simulink model "electrotac_feedback_emg_2016a"  (R2016a)
settings: Solver=FixedStepDiscrete  StartTime=0.0  StopTime=inf  FixedStep=0.02  RelTol=1e-3
undefined symbols (not defined in the file): DiscIntNeverNeededParam
libraries: PowermateLibrary x1, LIB_RehaMove3 x1, STIMYOLibrary x1
(part 2 of 3)

== stateflow chart electrotac_feedback_emg_2016a/stim_chart ==
  state preview
    state force_feedback1
      entry:
      reset_integrator = 0;
      during:
      stim_off_pw= [1 1 1 1];
      force_feedback_input = emg_value/12;
      state stim_n
        state stim_on
          during:
          pulsewidth = func.commonElectrode_4ch_stim(th_max,th_min,def_current,-def_current/4,0,'n','pw');
          current = func.commonElectrode_4ch_stim(th_max,th_min,def_current,-def_current/4,0,'n','cr');
          stim_status = func.commonElectrode_4ch_stim(th_max,th_min,def_current,-def_current/4,0,'n','lg');
          %ch3
        state stim_off [commented out]
          during:
          pulsewidth = func.commonElectrode_4ch_stim([0 0 0 0],th_min,def_current,-def_current/4,0,'e','pw');
          current = func.commonElectrode_4ch_stim([0 0 0 0],th_min,def_current,-def_current/4,0,'e','cr');
          %ch3
        (default) -> preview.force_feedback1.stim_n.stim_on
        preview.force_feedback1.stim_n.stim_on -> preview.force_feedback1.stim_n.stim_off [commented out] : after(input_freq,sec)
        preview.force_feedback1.stim_n.stim_off -> preview.force_feedback1.stim_n.stim_on [commented out] : after(input_freq,sec)
      state pos_nw6
        state stim_on
          during:
          pulsewidth = func.commonElectrode_4ch_stim(th_max,th_min,def_current,-def_current/4,0,'nw','pw');
          current = func.commonElectrode_4ch_stim(th_max,th_min,def_current,-def_current/4,0,'nw','cr');
          stim_status = func.commonElectrode_4ch_stim(th_max,th_min,def_current,-def_current/4,0,'nw','lg');
          %ch3
        state stim_off
          during:
          pulsewidth = func.commonElectrode_4ch_stim(stim_off_pw,th_min,def_current,-def_current/4,0,'nw','pw');
          current = func.commonElectrode_4ch_stim(stim_off_pw,th_min,def_current,-def_current/4,0,'nw','cr');
          stim_status = func.commonElectrode_4ch_stim(stim_off_pw,th_min,def_current,-def_current/4,0,'nw','lg');
          %ch3
        (default) -> preview.force_feedback1.pos_nw6.stim_on
        preview.force_feedback1.pos_nw6.stim_on -> preview.force_feedback1.pos_nw6.stim_off : after(0.2,sec)
        preview.force_feedback1.pos_nw6.stim_off -> preview.force_feedback1.pos_nw6.stim_on : after(0.2,sec)
      state pos_nw9
        state stim_on
          during:
          pulsewidth = func.commonElectrode_4ch_stim(th_max,th_min,def_current,-def_current/4,0,'ne','pw');
          current = func.commonElectrode_4ch_stim(th_max,th_min,def_current,-def_current/4,0,'ne','cr');
          stim_status = func.commonElectrode_4ch_stim(th_max,th_min,def_current,-def_current/4,0,'ne','lg');
          %ch3
        state stim_off
          during:
          pulsewidth = func.commonElectrode_4ch_stim(stim_off_pw,th_min,def_current,-def_current/4,0,'ne','pw');
          current = func.commonElectrode_4ch_stim(stim_off_pw,th_min,def_current,-def_current/4,0,'ne','cr');
          stim_status = func.commonElectrode_4ch_stim(stim_off_pw,th_min,def_current,-def_current/4,0,'ne','lg');
          %ch3
        (default) -> preview.force_feedback1.pos_nw9.stim_on
        preview.force_feedback1.pos_nw9.stim_on -> preview.force_feedback1.pos_nw9.stim_off : after(0.2,sec)
        preview.force_feedback1.pos_nw9.stim_off -> preview.force_feedback1.pos_nw9.stim_on : after(0.2,sec)
      state pos_nw10
        state stim_on
          during:
          pulsewidth = func.commonElectrode_4ch_stim(th_max,th_min,def_current,-def_current/4,0,'e','pw');
          current = func.commonElectrode_4ch_stim(th_max,th_min,def_current,-def_current/4,0,'e','cr');
          stim_status = func.commonElectrode_4ch_stim(th_max,th_min,def_current,-def_current/4,0,'e','lg');
          %ch3
        state stim_off [commented out]
          during:
          pulsewidth = func.commonElectrode_4ch_stim(stim_off_pw,th_min,def_current,-def_current/4,0,'e','pw');
          current = func.commonElectrode_4ch_stim(stim_off_pw,th_min,def_current,-def_current/4,0,'e','cr');
          stim_status = func.commonElectrode_4ch_stim(stim_off_pw,th_min,def_current,-def_current/4,0,'e','lg');
          %ch3
        (default) -> preview.force_feedback1.pos_nw10.stim_on
        preview.force_feedback1.pos_nw10.stim_on -> preview.force_feedback1.pos_nw10.stim_off [commented out] : after(0.2,sec)
        preview.force_feedback1.pos_nw10.stim_off -> preview.force_feedback1.pos_nw10.stim_on [commented out] : after(0.2,sec)
      state forcefeedback_3
        state stim_on
          during:
          pulsewidth = func.commonElectrode_4ch_stim(th_max,th_min,def_current,-def_current/4,0,'w','pw');
          current = func.commonElectrode_4ch_stim(th_max,th_min,def_current,-def_current/4,0,'w','cr');
          stim_status = func.commonElectrode_4ch_stim(th_max,th_min,def_current,-def_current/4,0,'w','lg');
          %ch3
        state stim_off [commented out]
          during:
          pulsewidth = func.commonElectrode_4ch_stim(stim_off_pw,th_min,def_current,-def_current/4,0,'nw','pw');
          current = func.commonElectrode_4ch_stim(stim_off_pw,th_min,def_current,-def_current/4,0,'nw','cr');
          stim_status = func.commonElectrode_4ch_stim(stim_off_pw,th_min,def_current,-def_current/4,0,'nw','lg');
          %ch3
        preview.force_feedback1.forcefeedback_3.stim_on -> preview.force_feedback1.forcefeedback_3.stim_off [commented out] : after(0.2,sec)
        preview.force_feedback1.forcefeedback_3.stim_off -> preview.force_feedback1.forcefeedback_3.stim_on [commented out] : after(0.2,sec)
      state forcefeedback_2
        state stim_on
          during:
          pulsewidth = func.commonElectrode_4ch_stim(th_max,th_min,def_current,-def_current/4,0,'w','pw');
          current = func.commonElectrode_4ch_stim(th_max,th_min,def_current,-def_current/4,0,'w','cr');
          stim_status = func.commonElectrode_4ch_stim(th_max,th_min,def_current,-def_current/4,0,'w','lg');
          %ch3
        state stim_off
          during:
          pulsewidth = func.commonElectrode_4ch_stim(stim_off_pw,th_min,def_current,-def_current/4,0,'w','pw');
          current = func.commonElectrode_4ch_stim(stim_off_pw,th_min,def_current,-def_current/4,0,'w','cr');
          stim_status = func.commonElectrode_4ch_stim(stim_off_pw,th_min,def_current,-def_current/4,0,'w','lg');
          %ch3
        (default) -> preview.force_feedback1.forcefeedback_2.stim_on
        preview.force_feedback1.forcefeedback_2.stim_on -> preview.force_feedback1.forcefeedback_2.stim_off : after(0.2,sec)
        preview.force_feedback1.forcefeedback_2.stim_off -> preview.force_feedback1.forcefeedback_2.stim_on : after(0.2,sec)
      state pos_nw11
        state stim_on
          during:
          pulsewidth = func.commonElectrode_4ch_stim(th_max,th_min,def_current,-def_current/4,0,'e','pw');
          current = func.commonElectrode_4ch_stim(th_max,th_min,def_current,-def_current/4,0,'e','cr');
          stim_status = func.commonElectrode_4ch_stim(th_max,th_min,def_current,-def_current/4,0,'e','lg');
          %ch3
        state stim_off
          during:
          pulsewidth = func.commonElectrode_4ch_stim(stim_off_pw,th_min,def_current,-def_current/4,0,'e','pw');
          current = func.commonElectrode_4ch_stim(stim_off_pw,th_min,def_current,-def_current/4,0,'e','cr');
          stim_status = func.commonElectrode_4ch_stim(stim_off_pw,th_min,def_current,-def_current/4,0,'e','lg');
          %ch3
        (default) -> preview.force_feedback1.pos_nw11.stim_on
        preview.force_feedback1.pos_nw11.stim_on -> preview.force_feedback1.pos_nw11.stim_off : after(0.2,sec)
        preview.force_feedback1.pos_nw11.stim_off -> preview.force_feedback1.pos_nw11.stim_on : after(0.2,sec)
      state stim_w
        state stim_on
          during:
          pulsewidth = func.commonElectrode_4ch_stim(th_max,th_min,def_current,-def_current/4,0,'sw','pw');
          current = func.commonElectrode_4ch_stim(th_max,th_min,def_current,-def_current/4,0,'sw','cr');
          stim_status = func.commonElectrode_4ch_stim(th_max,th_min,def_current,-def_current/4,0,'sw','lg');
          %ch3
        state stim_off
          during:
          pulsewidth = func.commonElectrode_4ch_stim(stim_off_pw,th_min,def_current,-def_current/4,0,'sw','pw');
          current = func.commonElectrode_4ch_stim(stim_off_pw,th_min,def_current,-def_current/4,0,'sw','cr');
          stim_status = func.commonElectrode_4ch_stim(stim_off_pw,th_min,def_current,-def_current/4,0,'sw','lg');
          %ch3
        (default) -> preview.force_feedback1.stim_w.stim_on
        preview.force_feedback1.stim_w.stim_on -> preview.force_feedback1.stim_w.stim_off : after(0.2,sec)
        preview.force_feedback1.stim_w.stim_off -> preview.force_feedback1.stim_w.stim_on : after(0.2,sec)
      state stim_e
        state stim_on
          during:
          pulsewidth = func.commonElectrode_4ch_stim(th_max,th_min,def_current,-def_current/4,0,'se','pw');
          current = func.commonElectrode_4ch_stim(th_max,th_min,def_current,-def_current/4,0,'se','cr');
          stim_status = func.commonElectrode_4ch_stim(th_max,th_min,def_current,-def_current/4,0,'se','lg');
          %ch3
        state stim_off
          during:
          pulsewidth = func.commonElectrode_4ch_stim(stim_off_pw,th_min,def_current,-def_current/4,0,'se','pw');
          current = func.commonElectrode_4ch_stim(stim_off_pw,th_min,def_current,-def_current/4,0,'se','cr');
          stim_status = func.commonElectrode_4ch_stim(stim_off_pw,th_min,def_current,-def_current/4,0,'se','lg');
          %ch3
        (default) -> preview.force_feedback1.stim_e.stim_on
        preview.force_feedback1.stim_e.stim_on -> preview.force_feedback1.stim_e.stim_off : after(0.2,sec)
        preview.force_feedback1.stim_e.stim_off -> preview.force_feedback1.stim_e.stim_on : after(0.2,sec)
      preview.force_feedback1.stim_n -> preview.force_feedback1.pos_nw9 : [c == 24]
      preview.force_feedback1.pos_nw6 -> preview.force_feedback1.stim_n : [c == 23]
      preview.force_feedback1.forcefeedback_3 -> preview.force_feedback1.pos_nw6 : [c == 22]
      preview.force_feedback1.pos_nw9 -> preview.force_feedback1.pos_nw10 : [c == 25]
      preview.force_feedback1.forcefeedback_2 -> preview.force_feedback1.forcefeedback_3 : [c == 21]
      preview.force_feedback1.pos_nw10 -> preview.force_feedback1.pos_nw11 : [c == 26]
      preview.force_feedback1.stim_w -> preview.force_feedback1.forcefeedback_2 : [c == 20]
      preview.force_feedback1.pos_nw11 -> preview.force_feedback1.stim_e : [c == 27]
      (default) -> preview.force_feedback1.stim_w
    state hand_openclosed1
      entry: reset_integrator = 0;
      during: stim_off_pw= [1 1 1 1]
      state neutral
        state pos_west2
          during:
          pulsewidth = func.commonElectrode_4ch_stim(stim_off_pw,th_min,def_current,-def_current/4,0,'ns','pw');
          current = func.commonElectrode_4ch_stim(stim_off_pw,th_min,def_current,-def_current/4,0,'ns','cr');
          stim_status = func.commonElectrode_4ch_stim(stim_off_pw,th_min,def_current,-def_current/4,0,'ns','lg');
          %ch3
      state level1
        state pos_west1
          during:
          pulsewidth = func.commonElectrode_4ch_stim(th_max,th_min,def_current,-def_current/4,0,'ns','pw');
          current = func.commonElectrode_4ch_stim(th_max,th_min,def_current,-def_current/4,0,'ns','cr');
          stim_status = func.commonElectrode_4ch_stim(th_max,th_min,def_current,-def_current/4,0,'ns','lg');
          %ch3
        state pos_west2
          during:
          pulsewidth = func.commonElectrode_4ch_stim(stim_off_pw,th_min,def_current,-def_current/4,0,'ns','pw');
          current = func.commonElectrode_4ch_stim(stim_off_pw,th_min,def_current,-def_current/4,0,'ns','cr');
          stim_status = func.commonElectrode_4ch_stim(stim_off_pw,th_min,def_current,-def_current/4,0,'ns','lg');
          %ch3
        (default) -> preview.hand_openclosed1.level1.pos_west1
        preview.hand_openclosed1.level1.pos_west1 -> preview.hand_openclosed1.level1.pos_west2 : after(0.5,sec)
        preview.hand_openclosed1.level1.pos_west2 -> preview.hand_openclosed1.level1.pos_west1 : after(0.5,sec)
      state level2
        state pos_west1
          during:
          pulsewidth = func.commonElectrode_4ch_stim(th_max,th_min,def_current,-def_current/4,0,'ns','pw');
          current = func.commonElectrode_4ch_stim(th_max,th_min,def_current,-def_current/4,0,'ns','cr');
          stim_status = func.commonElectrode_4ch_stim(th_max,th_min,def_current,-def_current/4,0,'ns','lg');
          %ch3
        state pos_west2
          during:
          pulsewidth = func.commonElectrode_4ch_stim(stim_off_pw,th_min,def_current,-def_current/4,0,'ns','pw');
          current = func.commonElectrode_4ch_stim(stim_off_pw,th_min,def_current,-def_current/4,0,'ns','cr');
          stim_status = func.commonElectrode_4ch_stim(stim_off_pw,th_min,def_current,-def_current/4,0,'ns','lg');
          %ch3
        (default) -> preview.hand_openclosed1.level2.pos_west1
        preview.hand_openclosed1.level2.pos_west1 -> preview.hand_openclosed1.level2.pos_west2 : after(0.25,sec)
        preview.hand_openclosed1.level2.pos_west2 -> preview.hand_openclosed1.level2.pos_west1 : after(0.25,sec)
      state level3
        state pos_west1
          during:
          pulsewidth = func.commonElectrode_4ch_stim(th_max,th_min,def_current,-def_current/4,0,'ns','pw');
          current = func.commonElectrode_4ch_stim(th_max,th_min,def_current,-def_current/4,0,'ns','cr');
          stim_status = func.commonElectrode_4ch_stim(th_max,th_min,def_current,-def_current/4,0,'ns','lg');
          %ch3
        (default) -> preview.hand_openclosed1.level3.pos_west1
      (default) -> preview.hand_openclosed1.neutral
      preview.hand_openclosed1.neutral -> preview.hand_openclosed1.level1 [order 1] : [c == 12]
      preview.hand_openclosed1.level1 -> preview.hand_openclosed1.neutral [order 2] : [c == 17]
      preview.hand_openclosed1.level1 -> preview.hand_openclosed1.level2 [order 1] : [c == 13]
      preview.hand_openclosed1.level2 -> preview.hand_openclosed1.level1 [order 2] : [c == 16]
      preview.hand_openclosed1.level2 -> preview.hand_openclosed1.level3 [order 1] : [c == 14]
      preview.hand_openclosed1.level3 -> preview.hand_openclosed1.level2 : [c == 15]
    state handposition_map2
      entry:
      reset_integrator = 0;
      during: stim_off_pw= [1 1 1 1]
      state pos_north_e2
        during:
        pulsewidth = func.commonElectrode_4ch_stim(th_max,th_min,def_current,-def_current/4,0,'n','pw');
        current = func.commonElectrode_4ch_stim(th_max,th_min,def_current,-def_current/4,0,'n','cr');
        stim_status = func.commonElectrode_4ch_stim(th_max,th_min,def_current,-def_current/4,0,'n','lg');
        %ch1
      state pos_nw1
        state pos_west1
          during:
          pulsewidth = func.commonElectrode_4ch_stim(th_max,th_min,def_current,-def_current/4,0,'ne','pw');
          current = func.commonElectrode_4ch_stim(th_max,th_min,def_current,-def_current/4,0,'ne','cr');
          stim_status = func.commonElectrode_4ch_stim(th_max,th_min,def_current,-def_current/4,0,'ne','lg');
          %ch3
        state pos_west2
          during:
          pulsewidth = func.commonElectrode_4ch_stim(stim_off_pw,th_min,def_current,-def_current/4,0,'ne','pw');
          current = func.commonElectrode_4ch_stim(stim_off_pw,th_min,def_current,-def_current/4,0,'ne','cr');
          stim_status = func.commonElectrode_4ch_stim(stim_off_pw,th_min,def_current,-def_current/4,0,'ne','lg');
          %ch3
        (default) -> preview.handposition_map2.pos_nw1.pos_west1
        preview.handposition_map2.pos_nw1.pos_west1 -> preview.handposition_map2.pos_nw1.pos_west2 : after(0.25,sec)
        preview.handposition_map2.pos_nw1.pos_west2 -> preview.handposition_map2.pos_nw1.pos_west1 : after(0.25,sec)
      state pos_nw
        state pos_west1
          during:
          pulsewidth = func.commonElectrode_4ch_stim(th_max,th_min,def_current,-def_current/4,0,'nw','pw');
          current = func.commonElectrode_4ch_stim(th_max,th_min,def_current,-def_current/4,0,'nw','cr');
          stim_status = func.commonElectrode_4ch_stim(th_max,th_min,def_current,-def_current/4,0,'nw','lg');
          %ch3
        state pos_west2
          during:
          pulsewidth = func.commonElectrode_4ch_stim(stim_off_pw,th_min,def_current,-def_current/4,0,'nw','pw');
          current = func.commonElectrode_4ch_stim(stim_off_pw,th_min,def_current,-def_current/4,0,'nw','cr');
          stim_status = func.commonElectrode_4ch_stim(stim_off_pw,th_min,def_current,-def_current/4,0,'nw','lg');
          %ch3
        (default) -> preview.handposition_map2.pos_nw.pos_west1
        preview.handposition_map2.pos_nw.pos_west1 -> preview.handposition_map2.pos_nw.pos_west2 : after(0.25,sec)
        preview.handposition_map2.pos_nw.pos_west2 -> preview.handposition_map2.pos_nw.pos_west1 : after(0.25,sec)
      state pos_west
        during:
        pulsewidth = func.commonElectrode_4ch_stim(th_max,th_min,def_current,-def_current/4,0,'w','pw');
        current = func.commonElectrode_4ch_stim(th_max,th_min,def_current,-def_current/4,0,'w','cr');
        stim_status = func.commonElectrode_4ch_stim(th_max,th_min,def_current,-def_current/4,0,'w','lg');
        %ch3
      state pos_east
        during:
        pulsewidth = func.commonElectrode_4ch_stim(th_max,th_min,def_current,-def_current/4,0,'e','pw');
        current = func.commonElectrode_4ch_stim(th_max,th_min,def_current,-def_current/4,0,'e','cr');
        stim_status = func.commonElectrode_4ch_stim(th_max,th_min,def_current,-def_current/4,0,'e','lg');
        %ch4
      state pos_nw2
        state pos_west1
          during:
          pulsewidth = func.commonElectrode_4ch_stim(th_max,th_min,def_current,-def_current/4,0,'sw','pw');
          current = func.commonElectrode_4ch_stim(th_max,th_min,def_current,-def_current/4,0,'sw','cr');
          stim_status = func.commonElectrode_4ch_stim(th_max,th_min,def_current,-def_current/4,0,'sw','lg');
          %ch3
        state pos_west2
          during:
          pulsewidth = func.commonElectrode_4ch_stim(stim_off_pw,th_min,def_current,-def_current/4,0,'sw','pw');
          current = func.commonElectrode_4ch_stim(stim_off_pw,th_min,def_current,-def_current/4,0,'sw','cr');
          stim_status = func.commonElectrode_4ch_stim(stim_off_pw,th_min,def_current,-def_current/4,0,'sw','lg');
          %ch3
        (default) -> preview.handposition_map2.pos_nw2.pos_west1
        preview.handposition_map2.pos_nw2.pos_west1 -> preview.handposition_map2.pos_nw2.pos_west2 : after(0.25,sec)
        preview.handposition_map2.pos_nw2.pos_west2 -> preview.handposition_map2.pos_nw2.pos_west1 : after(0.25,sec)
      state pos_nw3
        state pos_west1
          during:
          pulsewidth = func.commonElectrode_4ch_stim(th_max,th_min,def_current,-def_current/4,0,'se','pw');
          current = func.commonElectrode_4ch_stim(th_max,th_min,def_current,-def_current/4,0,'se','cr');
          stim_status = func.commonElectrode_4ch_stim(th_max,th_min,def_current,-def_current/4,0,'se','lg');
          %ch3
        state pos_west2
          during:
          pulsewidth = func.commonElectrode_4ch_stim(stim_off_pw,th_min,def_current,-def_current/4,0,'e','pw');
          current = func.commonElectrode_4ch_stim(stim_off_pw,th_min,def_current,-def_current/4,0,'e','cr');
          stim_status = func.commonElectrode_4ch_stim(stim_off_pw,th_min,def_current,-def_current/4,0,'e','lg');
          %ch3
        (default) -> preview.handposition_map2.pos_nw3.pos_west1
        preview.handposition_map2.pos_nw3.pos_west1 -> preview.handposition_map2.pos_nw3.pos_west2 : after(0.25,sec)
        preview.handposition_map2.pos_nw3.pos_west2 -> preview.handposition_map2.pos_nw3.pos_west1 : after(0.25,sec)
      state pos_south_e4
        during:
        pulsewidth = func.commonElectrode_4ch_stim(th_max,th_min,def_current,-def_current/4,0,'s','pw');
        current = func.commonElectrode_4ch_stim(th_max,th_min,def_current,-def_current/4,0,'s','cr');
        stim_status = func.commonElectrode_4ch_stim(th_max,th_min,def_current,-def_current/4,0,'s','lg');
        %ch2
      (default) -> preview.handposition_map2.pos_north_e2
      preview.handposition_map2.pos_north_e2 -> preview.handposition_map2.pos_nw : [c == 3]
      preview.handposition_map2.pos_east -> preview.handposition_map2.pos_nw1 : [c == 9]
      preview.handposition_map2.pos_nw -> preview.handposition_map2.pos_west : [c == 4]
      preview.handposition_map2.pos_west -> preview.handposition_map2.pos_nw2 : [c == 5]
      preview.handposition_map2.pos_nw3 -> preview.handposition_map2.pos_east : [c == 8]
      preview.handposition_map2.pos_nw2 -> preview.handposition_map2.pos_south_e4 : [c == 6]
      preview.handposition_map2.pos_south_e4 -> preview.handposition_map2.pos_nw3 : [c == 7]
    state NOP2
      entry:
      pulsewidth = func.commonElectrode_4ch_stim([0 0 0 0],th_min,def_current,-def_current/4,0,'we','pw');
      current = func.commonElectrode_4ch_stim([0 0 0 0],th_min,def_current,-def_current/4,0,'we','cr');
      stim_status = func.commonElectrode_4ch_stim([0 0 0 0],th_min,def_current,-def_current/4,0,'we','lg');
    state NOP1
      entry:
      pulsewidth = func.commonElectrode_4ch_stim([0 0 0 0],th_min,def_current,-def_current/4,0,'we','pw');
      current = func.commonElectrode_4ch_stim([0 0 0 0],th_min,def_current,-def_current/4,0,'we','cr');
      stim_status = func.commonElectrode_4ch_stim([0 0 0 0],th_min,def_current,-def_current/4,0,'we','lg');
    state jump6
    state jumplala
    state feedback_change_indicator6
      entry: jump_n = 0;
      state stim
        during:
        pulsewidth = func.commonElectrode_4ch_stim(th_max,th_min,def_current,-def_current/4,0,'we','pw');
        current = func.commonElectrode_4ch_stim(th_max,th_min,def_current,-def_current/4,0,'we','cr');
        stim_status = func.commonElectrode_4ch_stim(th_max,th_min,def_current,-def_current/4,0,'we','lg');
      state NOP
        entry:
        jump_n = jump_n + 1;
        pulsewidth = func.commonElectrode_4ch_stim([0 0 0 0],th_min,def_current,-def_current/4,0,'we','pw');
        current = func.commonElectrode_4ch_stim([0 0 0 0],th_min,def_current,-def_current/4,0,'we','cr');
        stim_status = func.commonElectrode_4ch_stim([0 0 0 0],th_min,def_current,-def_current/4,0,'we','lg');
      (default) -> preview.feedback_change_indicator6.stim
      preview.feedback_change_indicator6.stim -> preview.feedback_change_indicator6.NOP : after(0.25,sec)
      preview.feedback_change_indicator6.NOP -> preview.feedback_change_indicator6.stim [order 2] : after(0.25,sec)
    state feedback_change_indicator5
      entry: jump_n = 0;
      state stim
        during:
        pulsewidth = func.commonElectrode_4ch_stim(th_max,th_min,def_current,-def_current/4,0,'we','pw');
        current = func.commonElectrode_4ch_stim(th_max,th_min,def_current,-def_current/4,0,'we','cr');
        stim_status = func.commonElectrode_4ch_stim(th_max,th_min,def_current,-def_current/4,0,'we','lg');
      state NOP
        entry:
        jump_n = jump_n + 1;
        pulsewidth = func.commonElectrode_4ch_stim([0 0 0 0],th_min,def_current,-def_current/4,0,'we','pw');
        current = func.commonElectrode_4ch_stim([0 0 0 0],th_min,def_current,-def_current/4,0,'we','cr');
        stim_status = func.commonElectrode_4ch_stim([0 0 0 0],th_min,def_current,-def_current/4,0,'we','lg');
      (default) -> preview.feedback_change_indicator5.stim
      preview.feedback_change_indicator5.stim -> preview.feedback_change_indicator5.NOP : after(0.25,sec)
      preview.feedback_change_indicator5.NOP -> preview.feedback_change_indicator5.stim [order 2] : after(0.25,sec)
    state feedback_change_indicator4
      entry: jump_n = 0;
      state stim
        during:
        pulsewidth = func.commonElectrode_4ch_stim(th_max,th_min,def_current,-def_current/4,0,'we','pw');
        current = func.commonElectrode_4ch_stim(th_max,th_min,def_current,-def_current/4,0,'we','cr');
        stim_status = func.commonElectrode_4ch_stim(th_max,th_min,def_current,-def_current/4,0,'we','lg');
      state NOP
        entry:
        jump_n = jump_n + 1;
        pulsewidth = func.commonElectrode_4ch_stim([0 0 0 0],th_min,def_current,-def_current/4,0,'we','pw');
        current = func.commonElectrode_4ch_stim([0 0 0 0],th_min,def_current,-def_current/4,0,'we','cr');
        stim_status = func.commonElectrode_4ch_stim([0 0 0 0],th_min,def_current,-def_current/4,0,'we','lg');
      (default) -> preview.feedback_change_indicator4.stim
      preview.feedback_change_indicator4.stim -> preview.feedback_change_indicator4.NOP : after(0.25,sec)
      preview.feedback_change_indicator4.NOP -> preview.feedback_change_indicator4.stim [order 2] : after(0.25,sec)
    state jump5
    state NOP3
      entry:
      pulsewidth = func.commonElectrode_4ch_stim([0 0 0 0],th_min,def_current,-def_current/4,0,'we','pw');
      current = func.commonElectrode_4ch_stim([0 0 0 0],th_min,def_current,-def_current/4,0,'we','cr');
      stim_status = func.commonElectrode_4ch_stim([0 0 0 0],th_min,def_current,-def_current/4,0,'we','lg');
    state preview_on
    state preview_again
    state dummy2
    state duumy
    preview.hand_openclosed1.neutral -> NOP2 [order 2] : [c == 18]
    jump6 -> force_feedback1 : after(0.5,sec)[c == 19]
    jumplala -> hand_openclosed1 : after(0.5,sec)[c == 11]
    preview.handposition_map2.pos_nw1 -> NOP1 : [c == 10]
    preview.feedback_change_indicator6.NOP -> jump6 [order 1] : [jump_n == 3]
    NOP2 -> feedback_change_indicator6 : after(0.5,sec)
    NOP1 -> feedback_change_indicator5 : after(0.5,sec)
    preview.feedback_change_indicator5.NOP -> jumplala [order 1] : [jump_n == 2]
    jump5 -> handposition_map2 : after(0.5,sec)[c == 2]
    preview.feedback_change_indicator4.NOP -> jump5 [order 1] : [jump_n == 1]
    NOP3 -> preview.feedback_change_indicator4 : after(0.5,sec)
    preview_on -> NOP3 : [c == 1]
    (default) -> preview_on
    preview_again -> preview_on : [preview_again == 1]
    dummy2 -> preview_again
    preview.force_feedback1.stim_e -> duumy : [c == 28]
    duumy -> dummy2
  state func [group]
    note: ch1 - red, ch2 blue, ch3 black, ch4 white
    note: marked cable goes to common electrode
    note: ch1 - n, ch2 - s, ch3 - w, ch4 - e
  state testbench
    state stim_stop
      entry:
      pulsewidth = func.commonElectrode_4ch_emgstim([1 1 1 1],th_min,def_current,-def_current/4,0,'pw');
      current = func.commonElectrode_4ch_emgstim([1 1 1 1],th_min,def_current,-def_current/4,0,'cr');
      stim_status = func.commonElectrode_4ch_emgstim([1 1 1 1],th_min,def_current,-def_current/4,0,'lg');
    state stim_control
      entry:
      pulsewidth = func.commonElectrode_4ch_emgstim([1 1 1 1],th_min,def_current,-def_current/4,0,'pw');
      current = func.commonElectrode_4ch_emgstim([1 1 1 1],th_min,def_current,-def_current/4,0,'cr');
      stim_status = func.commonElectrode_4ch_emgstim([1 1 1 1],th_min,def_current,-def_current/4,0,'lg');
    state stim_stop3
      entry:
      pulsewidth = func.commonElectrode_4ch_emgstim([1 1 1 1],th_min,def_current,-def_current/4,0,'pw');
      current = func.commonElectrode_4ch_emgstim([1 1 1 1],th_min,def_current,-def_current/4,0,'cr');
      stim_status = func.commonElectrode_4ch_emgstim([1 1 1 1],th_min,def_current,-def_current/4,0,'lg');
    state feedback_change_indicator4
      entry: jump_n = 0;
      state stim
        during:
        pulsewidth = func.commonElectrode_4ch_stim(th_max,th_min,def_current,-def_current/4,0,'we','pw');
        current = func.commonElectrode_4ch_stim(th_max,th_min,def_current,-def_current/4,0,'we','cr');
        stim_status = func.commonElectrode_4ch_stim(th_max,th_min,def_current,-def_current/4,0,'we','lg');
      state NOP
        entry:
        pulsewidth = func.commonElectrode_4ch_stim([0 0 0 0],th_min,def_current,-def_current/4,0,'we','pw');
        current = func.commonElectrode_4ch_stim([0 0 0 0],th_min,def_current,-def_current/4,0,'we','cr');
        stim_status = func.commonElectrode_4ch_stim([0 0 0 0],th_min,def_current,-def_current/4,0,'we','lg');
        exit:
        jump_n = jump_n + 1;
      (default) -> testbench.feedback_change_indicator4.stim
      testbench.feedback_change_indicator4.stim -> testbench.feedback_change_indicator4.NOP : after(0.25,sec)
      testbench.feedback_change_indicator4.NOP -> testbench.feedback_change_indicator4.stim : after(0.25,sec)
    state handposition_map1
      entry:
      during: stim_off_pw= [1 1 1 1]
      exit:
      ready_for_stim = 0;
      state pos_north_e2
        entry:
        test_output = 1001;
        during:
        pulsewidth = func.commonElectrode_4ch_stim(th_max,th_min,def_current,-def_current/4,0,'n','pw');
        current = func.commonElectrode_4ch_stim(th_max,th_min,def_current,-def_current/4,0,'n','cr');
        stim_status = func.commonElectrode_4ch_stim(th_max,th_min,def_current,-def_current/4,0,'n','lg');
        %ch1
      state pos_nw
        entry: test_output = 1002;
        state pos_west1
          during:
          pulsewidth = func.commonElectrode_4ch_stim(th_max,th_min,def_current,-def_current/4,0,'nw','pw');
          current = func.commonElectrode_4ch_stim(th_max,th_min,def_current,-def_current/4,0,'nw','cr');
          stim_status = func.commonElectrode_4ch_stim(th_max,th_min,def_current,-def_current/4,0,'nw','lg');
          %ch3
        state pos_west2
          during:
          pulsewidth = func.commonElectrode_4ch_stim(stim_off_pw,th_min,def_current,-def_current/4,0,'nw','pw');
          current = func.commonElectrode_4ch_stim(stim_off_pw,th_min,def_current,-def_current/4,0,'nw','cr');
          stim_status = func.commonElectrode_4ch_stim(stim_off_pw,th_min,def_current,-def_current/4,0,'nw','lg');
          %ch3
        (default) -> testbench.handposition_map1.pos_nw.pos_west1
        testbench.handposition_map1.pos_nw.pos_west1 -> testbench.handposition_map1.pos_nw.pos_west2 : after(0.25,sec)
        testbench.handposition_map1.pos_nw.pos_west2 -> testbench.handposition_map1.pos_nw.pos_west1 : after(0.25,sec)
      state pos_nw1
        entry: test_output = 1008;
        state pos_west1
          during:
          pulsewidth = func.commonElectrode_4ch_stim(th_max,th_min,def_current,-def_current/4,0,'ne','pw');
          current = func.commonElectrode_4ch_stim(th_max,th_min,def_current,-def_current/4,0,'ne','cr');
          stim_status = func.commonElectrode_4ch_stim(th_max,th_min,def_current,-def_current/4,0,'ne','lg');
          %ch3
        state pos_west2
          during:
          pulsewidth = func.commonElectrode_4ch_stim(stim_off_pw,th_min,def_current,-def_current/4,0,'ne','pw');
          current = func.commonElectrode_4ch_stim(stim_off_pw,th_min,def_current,-def_current/4,0,'ne','cr');
          stim_status = func.commonElectrode_4ch_stim(stim_off_pw,th_min,def_current,-def_current/4,0,'ne','lg');
          %ch3
        (default) -> testbench.handposition_map1.pos_nw1.pos_west1
        testbench.handposition_map1.pos_nw1.pos_west1 -> testbench.handposition_map1.pos_nw1.pos_west2 : after(0.25,sec)
        testbench.handposition_map1.pos_nw1.pos_west2 -> testbench.handposition_map1.pos_nw1.pos_west1 : after(0.25,sec)
      state pos_west
        entry: test_output = 1003;
        during:
        pulsewidth = func.commonElectrode_4ch_stim(th_max,th_min,def_current,-def_current/4,0,'w','pw');
        current = func.commonElectrode_4ch_stim(th_max,th_min,def_current,-def_current/4,0,'w','cr');
        stim_status = func.commonElectrode_4ch_stim(th_max,th_min,def_current,-def_current/4,0,'w','lg');
        %ch3
      state pos_east
        entry: test_output = 1007;
        during:
        pulsewidth = func.commonElectrode_4ch_stim(th_max,th_min,def_current,-def_current/4,0,'e','pw');
        current = func.commonElectrode_4ch_stim(th_max,th_min,def_current,-def_current/4,0,'e','cr');
        stim_status = func.commonElectrode_4ch_stim(th_max,th_min,def_current,-def_current/4,0,'e','lg');
        %ch4
      state pos_nw2
        entry: test_output = 1004;
        state pos_west1
          during:
          pulsewidth = func.commonElectrode_4ch_stim(th_max,th_min,def_current,-def_current/4,0,'sw','pw');
          current = func.commonElectrode_4ch_stim(th_max,th_min,def_current,-def_current/4,0,'sw','cr');
          stim_status = func.commonElectrode_4ch_stim(th_max,th_min,def_current,-def_current/4,0,'sw','lg');
          %ch3
        state pos_west2
          during:
          pulsewidth = func.commonElectrode_4ch_stim(stim_off_pw,th_min,def_current,-def_current/4,0,'sw','pw');
          current = func.commonElectrode_4ch_stim(stim_off_pw,th_min,def_current,-def_current/4,0,'sw','cr');
          stim_status = func.commonElectrode_4ch_stim(stim_off_pw,th_min,def_current,-def_current/4,0,'sw','lg');
          %ch3
        (default) -> testbench.handposition_map1.pos_nw2.pos_west1
        testbench.handposition_map1.pos_nw2.pos_west1 -> testbench.handposition_map1.pos_nw2.pos_west2 : after(0.25,sec)
        testbench.handposition_map1.pos_nw2.pos_west2 -> testbench.handposition_map1.pos_nw2.pos_west1 : after(0.25,sec)
      state pos_nw3
        entry: test_output = 1006;
        state pos_west1
          during:
          pulsewidth = func.commonElectrode_4ch_stim(th_max,th_min,def_current,-def_current/4,0,'se','pw');
          current = func.commonElectrode_4ch_stim(th_max,th_min,def_current,-def_current/4,0,'se','cr');
          stim_status = func.commonElectrode_4ch_stim(th_max,th_min,def_current,-def_current/4,0,'se','lg');
          %ch3
        state pos_west2
          during:
          pulsewidth = func.commonElectrode_4ch_stim(stim_off_pw,th_min,def_current,-def_current/4,0,'e','pw');
          current = func.commonElectrode_4ch_stim(stim_off_pw,th_min,def_current,-def_current/4,0,'e','cr');
          stim_status = func.commonElectrode_4ch_stim(stim_off_pw,th_min,def_current,-def_current/4,0,'e','lg');
          %ch3
        (default) -> testbench.handposition_map1.pos_nw3.pos_west1
        testbench.handposition_map1.pos_nw3.pos_west1 -> testbench.handposition_map1.pos_nw3.pos_west2 : after(0.25,sec)
        testbench.handposition_map1.pos_nw3.pos_west2 -> testbench.handposition_map1.pos_nw3.pos_west1 : after(0.25,sec)
      state pos_south_e4
        entry: test_output = 1005;
        during:
        pulsewidth = func.commonElectrode_4ch_stim(th_max,th_min,def_current,-def_current/4,0,'s','pw');
        current = func.commonElectrode_4ch_stim(th_max,th_min,def_current,-def_current/4,0,'s','cr');
        stim_status = func.commonElectrode_4ch_stim(th_max,th_min,def_current,-def_current/4,0,'s','lg');
        %ch2
      (default) -> testbench.handposition_map1.pos_north_e2
      testbench.handposition_map1.pos_north_e2 -> testbench.handposition_map1.pos_nw : [test_value > 1.5]
      testbench.handposition_map1.pos_nw -> testbench.handposition_map1.pos_north_e2 [order 2] : [test_value < 1.5]
      testbench.handposition_map1.pos_nw -> testbench.handposition_map1.pos_west [order 1] : [test_value > 3]
      testbench.handposition_map1.pos_west -> testbench.handposition_map1.pos_nw [order 2] : [test_value < 3]
      testbench.handposition_map1.pos_nw1 -> testbench.handposition_map1.pos_east : [test_value < 10.5]
      testbench.handposition_map1.pos_east -> testbench.handposition_map1.pos_nw1 [order 1] : [test_value > 10.5]
      testbench.handposition_map1.pos_west -> testbench.handposition_map1.pos_nw2 [order 1] : [test_value > 4.5]
      testbench.handposition_map1.pos_nw2 -> testbench.handposition_map1.pos_west [order 2] : [test_value < 4.5]
      testbench.handposition_map1.pos_east -> testbench.handposition_map1.pos_nw3 [order 2] : [test_value < 9]
      testbench.handposition_map1.pos_nw3 -> testbench.handposition_map1.pos_east [order 1] : [test_value > 9]
      testbench.handposition_map1.pos_nw2 -> testbench.handposition_map1.pos_south_e4 [order 1] : [test_value > 6]
      testbench.handposition_map1.pos_south_e4 -> testbench.handposition_map1.pos_nw2 [order 2] : [test_value < 6]
      testbench.handposition_map1.pos_south_e4 -> testbench.handposition_map1.pos_nw3 [order 1] : [test_value > 7.5]
      testbench.handposition_map1.pos_nw3 -> testbench.handposition_map1.pos_south_e4 [order 2] : [test_value < 7.5]
    state force_feedback
      during:
      stim_off_pw= [1 1 1 1];
      test_force_feedback_input = test_value/12;
      exit: ready_for_stim = 0;
      state stim_n
        entry: test_output = 3005;
        state stim_on
          during:
          pulsewidth = func.commonElectrode_4ch_stim(th_max,th_min,def_current,-def_current/4,0,'n','pw');
          current = func.commonElectrode_4ch_stim(th_max,th_min,def_current,-def_current/4,0,'n','cr');
          stim_status = func.commonElectrode_4ch_stim(th_max,th_min,def_current,-def_current/4,0,'n','lg');
          %ch3
        state stim_off [commented out]
          during:
          pulsewidth = func.commonElectrode_4ch_stim([0 0 0 0],th_min,def_current,-def_current/4,0,'e','pw');
          current = func.commonElectrode_4ch_stim([0 0 0 0],th_min,def_current,-def_current/4,0,'e','cr');
          %ch3
        (default) -> testbench.force_feedback.stim_n.stim_on
        testbench.force_feedback.stim_n.stim_on -> testbench.force_feedback.stim_n.stim_off [commented out] : after(input_freq,sec)
        testbench.force_feedback.stim_n.stim_off -> testbench.force_feedback.stim_n.stim_on [commented out] : after(input_freq,sec)
      state pos_nw6
        entry: test_output = 3004;
        state stim_on
          during:
          pulsewidth = func.commonElectrode_4ch_stim(th_max,th_min,def_current,-def_current/4,0,'nw','pw');
          current = func.commonElectrode_4ch_stim(th_max,th_min,def_current,-def_current/4,0,'nw','cr');
          stim_status = func.commonElectrode_4ch_stim(th_max,th_min,def_current,-def_current/4,0,'nw','lg');
          %ch3
        state stim_off
          during:
          pulsewidth = func.commonElectrode_4ch_stim(stim_off_pw,th_min,def_current,-def_current/4,0,'nw','pw');
          current = func.commonElectrode_4ch_stim(stim_off_pw,th_min,def_current,-def_current/4,0,'nw','cr');
          stim_status = func.commonElectrode_4ch_stim(stim_off_pw,th_min,def_current,-def_current/4,0,'nw','lg');
          %ch3
        (default) -> testbench.force_feedback.pos_nw6.stim_on
        testbench.force_feedback.pos_nw6.stim_on -> testbench.force_feedback.pos_nw6.stim_off : after(0.2,sec)
        testbench.force_feedback.pos_nw6.stim_off -> testbench.force_feedback.pos_nw6.stim_on : after(0.2,sec)
      state pos_nw9
        entry: test_output = 3006;
        state stim_on
          during:
          pulsewidth = func.commonElectrode_4ch_stim(th_max,th_min,def_current,-def_current/4,0,'ne','pw');
          current = func.commonElectrode_4ch_stim(th_max,th_min,def_current,-def_current/4,0,'ne','cr');
          stim_status = func.commonElectrode_4ch_stim(th_max,th_min,def_current,-def_current/4,0,'ne','lg');
          %ch3
        state stim_off
          during:
          pulsewidth = func.commonElectrode_4ch_stim(stim_off_pw,th_min,def_current,-def_current/4,0,'ne','pw');
          current = func.commonElectrode_4ch_stim(stim_off_pw,th_min,def_current,-def_current/4,0,'ne','cr');
          stim_status = func.commonElectrode_4ch_stim(stim_off_pw,th_min,def_current,-def_current/4,0,'ne','lg');
          %ch3
        (default) -> testbench.force_feedback.pos_nw9.stim_on
        testbench.force_feedback.pos_nw9.stim_on -> testbench.force_feedback.pos_nw9.stim_off : after(0.2,sec)
        testbench.force_feedback.pos_nw9.stim_off -> testbench.force_feedback.pos_nw9.stim_on : after(0.2,sec)
      state pos_nw10
        entry: test_output = 3007;
        state stim_on
          during:
          pulsewidth = func.commonElectrode_4ch_stim(th_max,th_min,def_current,-def_current/4,0,'e','pw');
          current = func.commonElectrode_4ch_stim(th_max,th_min,def_current,-def_current/4,0,'e','cr');
          stim_status = func.commonElectrode_4ch_stim(th_max,th_min,def_current,-def_current/4,0,'e','lg');
          %ch3
        state stim_off [commented out]
          during:
          pulsewidth = func.commonElectrode_4ch_stim(stim_off_pw,th_min,def_current,-def_current/4,0,'e','pw');
          current = func.commonElectrode_4ch_stim(stim_off_pw,th_min,def_current,-def_current/4,0,'e','cr');
          stim_status = func.commonElectrode_4ch_stim(stim_off_pw,th_min,def_current,-def_current/4,0,'e','lg');
          %ch3
        (default) -> testbench.force_feedback.pos_nw10.stim_on
        testbench.force_feedback.pos_nw10.stim_on -> testbench.force_feedback.pos_nw10.stim_off [commented out] : after(0.2,sec)
        testbench.force_feedback.pos_nw10.stim_off -> testbench.force_feedback.pos_nw10.stim_on [commented out] : after(0.2,sec)
      state forcefeedback_3
        entry: test_output = 3003;
        state stim_on
          during:
          pulsewidth = func.commonElectrode_4ch_stim(th_max,th_min,def_current,-def_current/4,0,'w','pw');
          current = func.commonElectrode_4ch_stim(th_max,th_min,def_current,-def_current/4,0,'w','cr');
          stim_status = func.commonElectrode_4ch_stim(th_max,th_min,def_current,-def_current/4,0,'w','lg');
          %ch3
        state stim_off [commented out]
          during:
          pulsewidth = func.commonElectrode_4ch_stim(stim_off_pw,th_min,def_current,-def_current/4,0,'nw','pw');
          current = func.commonElectrode_4ch_stim(stim_off_pw,th_min,def_current,-def_current/4,0,'nw','cr');
          stim_status = func.commonElectrode_4ch_stim(stim_off_pw,th_min,def_current,-def_current/4,0,'nw','lg');
          %ch3
        (default) -> testbench.force_feedback.forcefeedback_3.stim_on
        testbench.force_feedback.forcefeedback_3.stim_on -> testbench.force_feedback.forcefeedback_3.stim_off [commented out] : after(0.2,sec)
        testbench.force_feedback.forcefeedback_3.stim_off -> testbench.force_feedback.forcefeedback_3.stim_on [commented out] : after(0.2,sec)
      state forcefeedback_2
        entry: test_output = 3002;
        state stim_on
          during:
          pulsewidth = func.commonElectrode_4ch_stim(th_max,th_min,def_current,-def_current/4,0,'w','pw');
          current = func.commonElectrode_4ch_stim(th_max,th_min,def_current,-def_current/4,0,'w','cr');
          stim_status = func.commonElectrode_4ch_stim(th_max,th_min,def_current,-def_current/4,0,'w','lg');
          %ch3
        state stim_off
          during:
          pulsewidth = func.commonElectrode_4ch_stim(stim_off_pw,th_min,def_current,-def_current/4,0,'w','pw');
          current = func.commonElectrode_4ch_stim(stim_off_pw,th_min,def_current,-def_current/4,0,'w','cr');
          stim_status = func.commonElectrode_4ch_stim(stim_off_pw,th_min,def_current,-def_current/4,0,'w','lg');
          %ch3
        (default) -> testbench.force_feedback.forcefeedback_2.stim_on
        testbench.force_feedback.forcefeedback_2.stim_on -> testbench.force_feedback.forcefeedback_2.stim_off : after(0.2,sec)
        testbench.force_feedback.forcefeedback_2.stim_off -> testbench.force_feedback.forcefeedback_2.stim_on : after(0.2,sec)
      state pos_nw11
        entry: test_output = 3008;
        state stim_on
          during:
          pulsewidth = func.commonElectrode_4ch_stim(th_max,th_min,def_current,-def_current/4,0,'e','pw');
          current = func.commonElectrode_4ch_stim(th_max,th_min,def_current,-def_current/4,0,'e','cr');
          stim_status = func.commonElectrode_4ch_stim(th_max,th_min,def_current,-def_current/4,0,'e','lg');
          %ch3
        state stim_off
          during:
          pulsewidth = func.commonElectrode_4ch_stim(stim_off_pw,th_min,def_current,-def_current/4,0,'e','pw');
          current = func.commonElectrode_4ch_stim(stim_off_pw,th_min,def_current,-def_current/4,0,'e','cr');
          stim_status = func.commonElectrode_4ch_stim(stim_off_pw,th_min,def_current,-def_current/4,0,'e','lg');
          %ch3
        (default) -> testbench.force_feedback.pos_nw11.stim_on
        testbench.force_feedback.pos_nw11.stim_on -> testbench.force_feedback.pos_nw11.stim_off : after(0.2,sec)
        testbench.force_feedback.pos_nw11.stim_off -> testbench.force_feedback.pos_nw11.stim_on : after(0.2,sec)
      state stim_w
        entry: test_output = 3001;
        state stim_on
          during:
          pulsewidth = func.commonElectrode_4ch_stim(th_max,th_min,def_current,-def_current/4,0,'sw','pw');
          current = func.commonElectrode_4ch_stim(th_max,th_min,def_current,-def_current/4,0,'sw','cr');
          stim_status = func.commonElectrode_4ch_stim(th_max,th_min,def_current,-def_current/4,0,'sw','lg');
          %ch3
        state stim_off
          during:
          pulsewidth = func.commonElectrode_4ch_stim(stim_off_pw,th_min,def_current,-def_current/4,0,'sw','pw');
          current = func.commonElectrode_4ch_stim(stim_off_pw,th_min,def_current,-def_current/4,0,'sw','cr');
          stim_status = func.commonElectrode_4ch_stim(stim_off_pw,th_min,def_current,-def_current/4,0,'sw','lg');
          %ch3
        (default) -> testbench.force_feedback.stim_w.stim_on
        testbench.force_feedback.stim_w.stim_on -> testbench.force_feedback.stim_w.stim_off : after(0.2,sec)
        testbench.force_feedback.stim_w.stim_off -> testbench.force_feedback.stim_w.stim_on : after(0.2,sec)
      state stim_e
        entry: test_output = 3009;
        state stim_on
          during:
          pulsewidth = func.commonElectrode_4ch_stim(th_max,th_min,def_current,-def_current/4,0,'se','pw');
          current = func.commonElectrode_4ch_stim(th_max,th_min,def_current,-def_current/4,0,'se','cr');
          stim_status = func.commonElectrode_4ch_stim(th_max,th_min,def_current,-def_current/4,0,'se','lg');
          %ch3
        state stim_off
          during:
          pulsewidth = func.commonElectrode_4ch_stim(stim_off_pw,th_min,def_current,-def_current/4,0,'se','pw');
          current = func.commonElectrode_4ch_stim(stim_off_pw,th_min,def_current,-def_current/4,0,'se','cr');
          stim_status = func.commonElectrode_4ch_stim(stim_off_pw,th_min,def_current,-def_current/4,0,'se','lg');
          %ch3
        (default) -> testbench.force_feedback.stim_e.stim_on
        testbench.force_feedback.stim_e.stim_on -> testbench.force_feedback.stim_e.stim_off : after(0.2,sec)
        testbench.force_feedback.stim_e.stim_off -> testbench.force_feedback.stim_e.stim_on : after(0.2,sec)
      (default) -> testbench.force_feedback.stim_n
      testbench.force_feedback.pos_nw9 -> testbench.force_feedback.stim_n [order 1] : [test_force_feedback_input <= 0.5625]
      testbench.force_feedback.stim_n -> testbench.force_feedback.pos_nw9 [order 2] : [test_force_feedback_input > 0.5625]
      testbench.force_feedback.stim_n -> testbench.force_feedback.pos_nw6 [order 1] : [test_force_feedback_input <= 0.4375]
      testbench.force_feedback.pos_nw6 -> testbench.force_feedback.stim_n [order 2] : [test_force_feedback_input > 0.4375]
      testbench.force_feedback.pos_nw6 -> testbench.force_feedback.forcefeedback_3 [order 1] : [test_force_feedback_input <= 0.3125]
      testbench.force_feedback.forcefeedback_3 -> testbench.force_feedback.pos_nw6 [order 2] : [test_force_feedback_input > 0.3125]
      testbench.force_feedback.pos_nw9 -> testbench.force_feedback.pos_nw10 [order 2] : [test_force_feedback_input > 0.6875]
      testbench.force_feedback.pos_nw10 -> testbench.force_feedback.pos_nw9 [order 1] : [test_force_feedback_input <= 0.6875]
      testbench.force_feedback.forcefeedback_3 -> testbench.force_feedback.forcefeedback_2 [order 1] : [test_force_feedback_input <= 0.1875]
      testbench.force_feedback.forcefeedback_2 -> testbench.force_feedback.forcefeedback_3 [order 1] : [test_force_feedback_input > 0.1875]
      testbench.force_feedback.pos_nw10 -> testbench.force_feedback.pos_nw11 [order 2] : [test_force_feedback_input > 0.8125]
      testbench.force_feedback.pos_nw11 -> testbench.force_feedback.pos_nw10 [order 1] : [test_force_feedback_input <= 0.8125]
      testbench.force_feedback.forcefeedback_2 -> testbench.force_feedback.stim_w [order 2] : [test_force_feedback_input <= 0.0625]
      testbench.force_feedback.stim_w -> testbench.force_feedback.forcefeedback_2 : [test_force_feedback_input > 0.0625]
      testbench.force_feedback.pos_nw11 -> testbench.force_feedback.stim_e [order 2] : [test_force_feedback_input > 0.9375]
      testbench.force_feedback.stim_e -> testbench.force_feedback.pos_nw11 : [test_force_feedback_input <= 0.9375]
    state stim_stop4
      entry:
      pulsewidth = func.commonElectrode_4ch_emgstim([1 1 1 1],th_min,def_current,-def_current/4,0,'pw');
      current = func.commonElectrode_4ch_emgstim([1 1 1 1],th_min,def_current,-def_current/4,0,'cr');
      stim_status = func.commonElectrode_4ch_emgstim([1 1 1 1],th_min,def_current,-def_current/4,0,'lg');
    state stim_pos
      during:
      pulsewidth = func.commonElectrode_4ch_pos(th_max, th_min, def_current, -def_current/4, 0, test_value*30, 'pw');
      current = func.commonElectrode_4ch_pos(th_max, th_min, def_current, -def_current/4, 0, test_value*30, 'cr');
      stim_status = func.commonElectrode_4ch_pos(th_max, th_min, def_current, -def_current/4, 0, test_value*30, 'lg');
      test_output = test_value*30;
      exit:ready_for_stim = 0;
    state stim_stop2
      entry:
      pulsewidth = func.commonElectrode_4ch_emgstim([1 1 1 1],th_min,def_current,-def_current/4,0,'pw');
      current = func.commonElectrode_4ch_emgstim([1 1 1 1],th_min,def_current,-def_current/4,0,'cr');
      stim_status = func.commonElectrode_4ch_emgstim([1 1 1 1],th_min,def_current,-def_current/4,0,'lg');
    state hand_openclosed
      during: stim_off_pw= [1 1 1 1]
      exit:ready_for_stim = 0;
      state neutral
        entry: test_output = 2001;
        state pos_west2
          during:
          pulsewidth = func.commonElectrode_4ch_stim(stim_off_pw,th_min,def_current,-def_current/4,0,'ns','pw');
          current = func.commonElectrode_4ch_stim(stim_off_pw,th_min,def_current,-def_current/4,0,'ns','cr');
          stim_status = func.commonElectrode_4ch_stim(stim_off_pw,th_min,def_current,-def_current/4,0,'ns','lg');
          %ch3
      state level1
        entry: user_output = 2002;
        state pos_west1
          during:
          pulsewidth = func.commonElectrode_4ch_stim(th_max,th_min,def_current,-def_current/4,0,'ns','pw');
          current = func.commonElectrode_4ch_stim(th_max,th_min,def_current,-def_current/4,0,'ns','cr');
          stim_status = func.commonElectrode_4ch_stim(th_max,th_min,def_current,-def_current/4,0,'ns','lg');
          %ch3
        state pos_west2
          during:
          pulsewidth = func.commonElectrode_4ch_stim(stim_off_pw,th_min,def_current,-def_current/4,0,'ns','pw');
          current = func.commonElectrode_4ch_stim(stim_off_pw,th_min,def_current,-def_current/4,0,'ns','cr');
          stim_status = func.commonElectrode_4ch_stim(stim_off_pw,th_min,def_current,-def_current/4,0,'ns','lg');
          %ch3
        (default) -> testbench.hand_openclosed.level1.pos_west1
        testbench.hand_openclosed.level1.pos_west1 -> testbench.hand_openclosed.level1.pos_west2 : after(0.5,sec)
        testbench.hand_openclosed.level1.pos_west2 -> testbench.hand_openclosed.level1.pos_west1 : after(0.5,sec)
      state level2
        entry:  test_output = 2003;
        state pos_west1
          during:
          pulsewidth = func.commonElectrode_4ch_stim(th_max,th_min,def_current,-def_current/4,0,'ns','pw');
          current = func.commonElectrode_4ch_stim(th_max,th_min,def_current,-def_current/4,0,'ns','cr');
          stim_status = func.commonElectrode_4ch_stim(th_max,th_min,def_current,-def_current/4,0,'ns','lg');
          %ch3
        state pos_west2
          during:
          pulsewidth = func.commonElectrode_4ch_stim(stim_off_pw,th_min,def_current,-def_current/4,0,'ns','pw');
          current = func.commonElectrode_4ch_stim(stim_off_pw,th_min,def_current,-def_current/4,0,'ns','cr');
          stim_status = func.commonElectrode_4ch_stim(stim_off_pw,th_min,def_current,-def_current/4,0,'ns','lg');
          %ch3
        (default) -> testbench.hand_openclosed.level2.pos_west1
        testbench.hand_openclosed.level2.pos_west1 -> testbench.hand_openclosed.level2.pos_west2 : after(0.25,sec)
        testbench.hand_openclosed.level2.pos_west2 -> testbench.hand_openclosed.level2.pos_west1 : after(0.25,sec)
      state level3
        entry:  test_output = 2004;
        state pos_west1
          during:
          pulsewidth = func.commonElectrode_4ch_stim(th_max,th_min,def_current,-def_current/4,0,'ns','pw');
          current = func.commonElectrode_4ch_stim(th_max,th_min,def_current,-def_current/4,0,'ns','cr');
          stim_status = func.commonElectrode_4ch_stim(th_max,th_min,def_current,-def_current/4,0,'ns','lg');
          %ch3
        (default) -> testbench.hand_openclosed.level3.pos_west1
      (default) -> testbench.hand_openclosed.neutral
      testbench.hand_openclosed.neutral -> testbench.hand_openclosed.level1 : [test_value >= 3]
      testbench.hand_openclosed.level1 -> testbench.hand_openclosed.neutral [order 2] : [test_value < 3]
      testbench.hand_openclosed.level1 -> testbench.hand_openclosed.level2 [order 1] : [test_value >= 6]
      testbench.hand_openclosed.level2 -> testbench.hand_openclosed.level1 [order 2] : [test_value < 6]
      testbench.hand_openclosed.level2 -> testbench.hand_openclosed.level3 [order 1] : [test_value >= 9]
      testbench.hand_openclosed.level3 -> testbench.hand_openclosed.level2 : [test_value < 9]
    (default) -> testbench.stim_control
    testbench.feedback_change_indicator4 -> stim_stop3 [order 3] : [jump_n == test_command && test_command == 3]{ready_for_stim = 1}
    stim_stop -> testbench.handposition_map1 : after(0.5,sec)
    testbench.feedback_change_indicator4 -> stim_stop [order 1] : [jump_n == test_command && test_command == 1]{ready_for_stim = 1}
    testbench.hand_openclosed -> testbench.stim_control : [test_command ~= 2]
    testbench.force_feedback -> testbench.stim_control : [test_command ~= 3]
    testbench.handposition_map1 -> testbench.stim_control : [test_command ~= 1]
    testbench.stim_pos -> testbench.stim_control : [test_command ~= 4]
    testbench.stim_control -> testbench.feedback_change_indicator4 : after(0.5,sec)[test_command ~= 0]
    stim_stop3 -> testbench.force_feedback : after(0.5,sec)
    testbench.feedback_change_indicator4 -> stim_stop4 [order 4] : [jump_n == test_command && test_command == 4]{ready_for_stim = 1}
    stim_stop4 -> testbench.stim_pos : after(0.5,sec)
    testbench.feedback_change_indicator4 -> stim_stop2 [order 2] : [jump_n == test_command && test_command == 2]{ready_for_stim = 1}
    stim_stop2 -> testbench.hand_openclosed : after(0.5,sec)
  state threshold_val_max_ch1
    during:
    pulsewidth = func.commonElectrode_4ch_threshold(value_pw+1, def_current, -def_current/4, 0, 1, 'pw');
    current = func.commonElectrode_4ch_threshold(value_pw+1, def_current, -def_current/4, 0, 1, 'cr');
    stim_status = func.commonElectrode_4ch_threshold(value_pw+1, def_current, -def_current/4, 0, 1, 'lg');
  state threshold_val_min_ch1
    during:
    pulsewidth = func.commonElectrode_4ch_threshold(value_pw+1, def_current, -def_current/4, 0, 1, 'pw');
    current = func.commonElectrode_4ch_threshold(value_pw+1, def_current, -def_current/4, 0, 1, 'cr');
    stim_status = func.commonElectrode_4ch_threshold(value_pw+1,def_current, -def_current/4, 0, 1, 'lg');
  state init
    entry:
    value_pw;
    single_click;
    def_current;
    th_max;
    th_min;
  state threshold_val_min_ch2
    during:
    pulsewidth = func.commonElectrode_4ch_threshold(value_pw+1, def_current, -def_current/4, 0, 2, 'pw');
    current = func.commonElectrode_4ch_threshold(value_pw+1, def_current, -def_current/4, 0, 2, 'cr');
    stim_status = func.commonElectrode_4ch_threshold(value_pw+1, def_current, -def_current/4, 0, 2, 'lg');
  state threshold_val_max_ch2
    during:
    pulsewidth = func.commonElectrode_4ch_threshold(value_pw+1, def_current, -def_current/4, 0, 2, 'pw');
    current = func.commonElectrode_4ch_threshold(value_pw+1, def_current, -def_current/4, 0, 2, 'cr');
    stim_status = func.commonElectrode_4ch_threshold(value_pw+1, def_current, -def_current/4, 0, 2, 'lg');
  state threshold_val_min_ch3
    during:
    pulsewidth = func.commonElectrode_4ch_threshold(value_pw+1, def_current, -def_current/4, 0, 3, 'pw');
    current = func.commonElectrode_4ch_threshold(value_pw+1, def_current, -def_current/4, 0, 3, 'cr');
    stim_status = func.commonElectrode_4ch_threshold(value_pw+1, def_current, -def_current/4, 0, 3, 'lg');
  state threshold_val_max_ch3
    during:
    pulsewidth = func.commonElectrode_4ch_threshold(value_pw+1, def_current, -def_current/4, 0, 3, 'pw');
    current = func.commonElectrode_4ch_threshold(value_pw+1, def_current, -def_current/4, 0, 3, 'cr');
    stim_status = func.commonElectrode_4ch_threshold(value_pw+1, def_current, -def_current/4, 0, 3, 'lg');
  state threshold_val_max_ch4
    during:
    pulsewidth = func.commonElectrode_4ch_threshold(value_pw+1, def_current, -def_current/4, 0, 4, 'pw');
    current = func.commonElectrode_4ch_threshold(value_pw+1, def_current, -def_current/4, 0, 4, 'cr');
    stim_status = func.commonElectrode_4ch_threshold(value_pw+1, def_current, -def_current/4, 0, 4, 'lg');
  state threshold_val_min_ch4
    during:
    pulsewidth = func.commonElectrode_4ch_threshold(value_pw+1, def_current, -def_current/4, 0, 4, 'pw');
    current = func.commonElectrode_4ch_threshold(value_pw+1, def_current, -def_current/4, 0, 4, 'cr');
    stim_status = func.commonElectrode_4ch_threshold(value_pw+1, def_current, -def_current/4, 0, 4, 'lg');
  state stimfor_emg_thresholds
    state stimfor_emg_ch1
      during:
      pulsewidth = func.commonElectrode_4ch_emgstim(th_min,th_min,def_current,-def_current/4,0,'pw');
      current = func.commonElectrode_4ch_emgstim(th_min,th_min,def_current,-def_current/4,0,'cr');
      stim_status = func.commonElectrode_4ch_emgstim(th_min,th_min,def_current,-def_current/4,0,'lg');
    state stop
      during:
      pulsewidth = func.commonElectrode_4ch_emgstim([1 1 1 1],th_min,def_current,-def_current/4,0,'pw');
      current = func.commonElectrode_4ch_emgstim([1 1 1 1],th_min,def_current,-def_current/4,0,'cr');
      stim_status = func.commonElectrode_4ch_emgstim([1 1 1 1],th_min,def_current,-def_current/4,0,'lg');
    state stimfor_emg_ch2
      during:
      pulsewidth = func.commonElectrode_4ch_emgstim(th_min,th_min,def_current,-def_current/4,0,'pw');
      current = func.commonElectrode_4ch_emgstim(th_min,th_min,def_current,-def_current/4,0,'cr');
      stim_status = func.commonElectrode_4ch_emgstim(th_min,th_min,def_current,-def_current/4,0,'lg');
    state stop2
      during:
      pulsewidth = func.commonElectrode_4ch_emgstim([1 1 1 1],th_min,def_current,-def_current/4,0,'pw');
      current = func.commonElectrode_4ch_emgstim([1 1 1 1],th_min,def_current,-def_current/4,0,'cr');
      stim_status = func.commonElectrode_4ch_emgstim([1 1 1 1],th_min,def_current,-def_current/4,0,'lg');
    (default) -> stimfor_emg_ch1
    stimfor_emg_ch1 -> stop : [n == 10]
    stop -> stimfor_emg_ch2 : [n == 11]
    stimfor_emg_ch2 -> stop2 : [n == 12]
  state stim_opcl [commented out]
    entry:
    reset_integrator = 0;
    during:
    pulsewidth = func.commonElectrode_4ch_opcl(th_max, th_min, def_current, -def_current/4, 0, emg_value_zeroed,12, 'pw');
    current = func.commonElectrode_4ch_opcl(th_max, th_min, def_current, -def_current/4, 0, emg_value_zeroed,12, 'cr');
    stim_status = func.commonElectrode_4ch_opcl(th_max, th_min, def_current, -def_current/4, 0, emg_value_zeroed,12, 'lg');
    user_output = emg_value_zeroed;
  state stim_forcefeedback [commented out]
    entry:
    reset_integrator = 0;
    during:
    pulsewidth = func.commonElectrode_4ch_forcefeedback(th_max, th_min, def_current, -def_current/4, 0, emg_value,12, 'pw');
    current = func.commonElectrode_4ch_forcefeedback(th_max, th_min, def_current, -def_current/4, 0, emg_value,12, 'cr');
    stim_status = func.commonElectrode_4ch_forcefeedback(th_max, th_min, def_current, -def_current/4, 0, emg_value,12, 'lg');
    user_output = emg_value;
  state selection
    entry:
    pulsewidth = func.commonElectrode_4ch_emgstim([1 1 1 1],th_min,def_current,-def_current/4,0,'pw');
    current = func.commonElectrode_4ch_emgstim([1 1 1 1],th_min,def_current,-def_current/4,0,'cr');
    stim_status = func.commonElectrode_4ch_emgstim([1 1 1 1],th_min,def_current,-def_current/4,0,'lg');
    return_pos = 0;
    return_opcl = 0;
    return_force = 0;
    return_cont_pos = 0;
  state freeform_chart
    state wait
      entry: pulsewidth = func.commonElectrode_4ch_emgstim([1 1 1 1],th_min,def_current,-def_current/4,0,'pw');
      current = func.commonElectrode_4ch_emgstim([1 1 1 1],th_min,def_current,-def_current/4,0,'cr');
      stim_status = func.commonElectrode_4ch_emgstim([1 1 1 1],th_min,def_current,-def_current/4,0,'lg');
    state stim_control
      entry:
      pulsewidth = func.commonElectrode_4ch_emgstim([1 1 1 1],th_min,def_current,-def_current/4,0,'pw');
      current = func.commonElectrode_4ch_emgstim([1 1 1 1],th_min,def_current,-def_current/4,0,'cr');
      stim_status = func.commonElectrode_4ch_emgstim([1 1 1 1],th_min,def_current,-def_current/4,0,'lg');
    state wait4
    state disc_pos
      entry:
      init_for_integrator = return_pos;
    state disc_force
      entry:
      init_for_integrator = return_force;
    state wait2
      entry: pulsewidth = func.commonElectrode_4ch_emgstim([1 1 1 1],th_min,def_current,-def_current/4,0,'pw');
      current = func.commonElectrode_4ch_emgstim([1 1 1 1],th_min,def_current,-def_current/4,0,'cr');
      stim_status = func.commonElectrode_4ch_emgstim([1 1 1 1],th_min,def_current,-def_current/4,0,'lg');
    state wait7
    state feedback_change_indicator4
      entry: jump_n = 0;
      state stim
        during:
        pulsewidth = func.commonElectrode_4ch_stim(th_max,th_min,def_current,-def_current/4,0,'we','pw');
        current = func.commonElectrode_4ch_stim(th_max,th_min,def_current,-def_current/4,0,'we','cr');
        stim_status = func.commonElectrode_4ch_stim(th_max,th_min,def_current,-def_current/4,0,'we','lg');
      state NOP
        entry:
        pulsewidth = func.commonElectrode_4ch_stim([0 0 0 0],th_min,def_current,-def_current/4,0,'we','pw');
        current = func.commonElectrode_4ch_stim([0 0 0 0],th_min,def_current,-def_current/4,0,'we','cr');
        stim_status = func.commonElectrode_4ch_stim([0 0 0 0],th_min,def_current,-def_current/4,0,'we','lg');
        exit:
        jump_n = jump_n + 1;
      (default) -> freeform_chart.feedback_change_indicator4.stim
      freeform_chart.feedback_change_indicator4.stim -> freeform_chart.feedback_change_indicator4.NOP : after(0.25,sec)
      freeform_chart.feedback_change_indicator4.NOP -> freeform_chart.feedback_change_indicator4.stim : after(0.25,sec)
    state handposition_map1
      entry:
      reset_integrator = 0;
      during: stim_off_pw= [1 1 1 1]
      state pos_north_e2
        entry:
        return_pos = 0;
        user_output = 1001;
        during:
        pulsewidth = func.commonElectrode_4ch_stim(th_max,th_min,def_current,-def_current/4,0,'n','pw');
        current = func.commonElectrode_4ch_stim(th_max,th_min,def_current,-def_current/4,0,'n','cr');
        stim_status = func.commonElectrode_4ch_stim(th_max,th_min,def_current,-def_current/4,0,'n','lg');
        %ch1
      state pos_nw
        entry: user_output = 1002;
        return_pos = 2.25;
        state pos_west1
          during:
          pulsewidth = func.commonElectrode_4ch_stim(th_max,th_min,def_current,-def_current/4,0,'nw','pw');
          current = func.commonElectrode_4ch_stim(th_max,th_min,def_current,-def_current/4,0,'nw','cr');
          stim_status = func.commonElectrode_4ch_stim(th_max,th_min,def_current,-def_current/4,0,'nw','lg');
          %ch3
        state pos_west2
          during:
          pulsewidth = func.commonElectrode_4ch_stim(stim_off_pw,th_min,def_current,-def_current/4,0,'nw','pw');
          current = func.commonElectrode_4ch_stim(stim_off_pw,th_min,def_current,-def_current/4,0,'nw','cr');
          stim_status = func.commonElectrode_4ch_stim(stim_off_pw,th_min,def_current,-def_current/4,0,'nw','lg');
          %ch3
        (default) -> freeform_chart.handposition_map1.pos_nw.pos_west1
        freeform_chart.handposition_map1.pos_nw.pos_west1 -> freeform_chart.handposition_map1.pos_nw.pos_west2 : after(0.25,sec)
        freeform_chart.handposition_map1.pos_nw.pos_west2 -> freeform_chart.handposition_map1.pos_nw.pos_west1 : after(0.25,sec)
      state pos_nw1
        entry: user_output = 1008;
        return_pos = 12;
        state pos_west1
          during:
          pulsewidth = func.commonElectrode_4ch_stim(th_max,th_min,def_current,-def_current/4,0,'ne','pw');
          current = func.commonElectrode_4ch_stim(th_max,th_min,def_current,-def_current/4,0,'ne','cr');
          stim_status = func.commonElectrode_4ch_stim(th_max,th_min,def_current,-def_current/4,0,'ne','lg');
          %ch3
        state pos_west2
          during:
          pulsewidth = func.commonElectrode_4ch_stim(stim_off_pw,th_min,def_current,-def_current/4,0,'ne','pw');
          current = func.commonElectrode_4ch_stim(stim_off_pw,th_min,def_current,-def_current/4,0,'ne','cr');
          stim_status = func.commonElectrode_4ch_stim(stim_off_pw,th_min,def_current,-def_current/4,0,'ne','lg');
          %ch3
        (default) -> freeform_chart.handposition_map1.pos_nw1.pos_west1
        freeform_chart.handposition_map1.pos_nw1.pos_west1 -> freeform_chart.handposition_map1.pos_nw1.pos_west2 : after(0.25,sec)
        freeform_chart.handposition_map1.pos_nw1.pos_west2 -> freeform_chart.handposition_map1.pos_nw1.pos_west1 : after(0.25,sec)
      state pos_west
        entry: user_output = 1003;
        return_pos = 3.5;
        during:
        pulsewidth = func.commonElectrode_4ch_stim(th_max,th_min,def_current,-def_current/4,0,'w','pw');
        current = func.commonElectrode_4ch_stim(th_max,th_min,def_current,-def_current/4,0,'w','cr');
        stim_status = func.commonElectrode_4ch_stim(th_max,th_min,def_current,-def_current/4,0,'w','lg');
        %ch3
      state pos_east
        entry: user_output = 1007;
        return_pos  = 9.75;
        during:
        pulsewidth = func.commonElectrode_4ch_stim(th_max,th_min,def_current,-def_current/4,0,'e','pw');
        current = func.commonElectrode_4ch_stim(th_max,th_min,def_current,-def_current/4,0,'e','cr');
        stim_status = func.commonElectrode_4ch_stim(th_max,th_min,def_current,-def_current/4,0,'e','lg');
        %ch4
      state pos_nw2
        entry: user_output = 1004;
        return_pos = 5.25;
        state pos_west1
          during:
          pulsewidth = func.commonElectrode_4ch_stim(th_max,th_min,def_current,-def_current/4,0,'sw','pw');
          current = func.commonElectrode_4ch_stim(th_max,th_min,def_current,-def_current/4,0,'sw','cr');
          stim_status = func.commonElectrode_4ch_stim(th_max,th_min,def_current,-def_current/4,0,'sw','lg');
          %ch3
        state pos_west2
          during:
          pulsewidth = func.commonElectrode_4ch_stim(stim_off_pw,th_min,def_current,-def_current/4,0,'sw','pw');
          current = func.commonElectrode_4ch_stim(stim_off_pw,th_min,def_current,-def_current/4,0,'sw','cr');
          stim_status = func.commonElectrode_4ch_stim(stim_off_pw,th_min,def_current,-def_current/4,0,'sw','lg');
          %ch3
        (default) -> freeform_chart.handposition_map1.pos_nw2.pos_west1
        freeform_chart.handposition_map1.pos_nw2.pos_west1 -> freeform_chart.handposition_map1.pos_nw2.pos_west2 : after(0.25,sec)
        freeform_chart.handposition_map1.pos_nw2.pos_west2 -> freeform_chart.handposition_map1.pos_nw2.pos_west1 : after(0.25,sec)
      state pos_nw3
        entry: user_output = 1006;
        return_pos = 8.25;
        state pos_west1
          during:
          pulsewidth = func.commonElectrode_4ch_stim(th_max,th_min,def_current,-def_current/4,0,'se','pw');
          current = func.commonElectrode_4ch_stim(th_max,th_min,def_current,-def_current/4,0,'se','cr');
          stim_status = func.commonElectrode_4ch_stim(th_max,th_min,def_current,-def_current/4,0,'se','lg');
          %ch3
        state pos_west2
          during:
          pulsewidth = func.commonElectrode_4ch_stim(stim_off_pw,th_min,def_current,-def_current/4,0,'e','pw');
          current = func.commonElectrode_4ch_stim(stim_off_pw,th_min,def_current,-def_current/4,0,'e','cr');
          stim_status = func.commonElectrode_4ch_stim(stim_off_pw,th_min,def_current,-def_current/4,0,'e','lg');
          %ch3
        (default) -> freeform_chart.handposition_map1.pos_nw3.pos_west1
        freeform_chart.handposition_map1.pos_nw3.pos_west1 -> freeform_chart.handposition_map1.pos_nw3.pos_west2 : after(0.25,sec)
        freeform_chart.handposition_map1.pos_nw3.pos_west2 -> freeform_chart.handposition_map1.pos_nw3.pos_west1 : after(0.25,sec)
      state pos_south_e4
        entry: user_output = 1005;
        return_pos = 6.5;
        during:
        pulsewidth = func.commonElectrode_4ch_stim(th_max,th_min,def_current,-def_current/4,0,'s','pw');
        current = func.commonElectrode_4ch_stim(th_max,th_min,def_current,-def_current/4,0,'s','cr');
        stim_status = func.commonElectrode_4ch_stim(th_max,th_min,def_current,-def_current/4,0,'s','lg');
        %ch2
      (default) -> freeform_chart.handposition_map1.pos_north_e2
      freeform_chart.handposition_map1.pos_north_e2 -> freeform_chart.handposition_map1.pos_nw : [emg_value > 1.5]
      freeform_chart.handposition_map1.pos_nw -> freeform_chart.handposition_map1.pos_north_e2 [order 2] : [emg_value < 1.5]
      freeform_chart.handposition_map1.pos_west -> freeform_chart.handposition_map1.pos_nw [order 2] : [emg_value < 3]
      freeform_chart.handposition_map1.pos_nw -> freeform_chart.handposition_map1.pos_west [order 1] : [emg_value > 3]
      freeform_chart.handposition_map1.pos_nw1 -> freeform_chart.handposition_map1.pos_east : [emg_value < 10.5]
      freeform_chart.handposition_map1.pos_east -> freeform_chart.handposition_map1.pos_nw1 [order 1] : [emg_value > 10.5]
      freeform_chart.handposition_map1.pos_west -> freeform_chart.handposition_map1.pos_nw2 [order 1] : [emg_value > 4.5]
      freeform_chart.handposition_map1.pos_nw2 -> freeform_chart.handposition_map1.pos_west [order 2] : [emg_value < 4.5]
      freeform_chart.handposition_map1.pos_east -> freeform_chart.handposition_map1.pos_nw3 [order 2] : [emg_value < 9]
      freeform_chart.handposition_map1.pos_nw3 -> freeform_chart.handposition_map1.pos_east [order 1] : [emg_value > 9]
      freeform_chart.handposition_map1.pos_nw2 -> freeform_chart.handposition_map1.pos_south_e4 [order 1] : [emg_value > 6]
      freeform_chart.handposition_map1.pos_south_e4 -> freeform_chart.handposition_map1.pos_nw2 [order 2] : [emg_value < 6]
      freeform_chart.handposition_map1.pos_south_e4 -> freeform_chart.handposition_map1.pos_nw3 [order 1] : [emg_value > 7.5]
      freeform_chart.handposition_map1.pos_nw3 -> freeform_chart.handposition_map1.pos_south_e4 [order 2] : [emg_value < 7.5]
    state force_feedback
      entry:
      reset_integrator = 0;
      during:
      stim_off_pw= [1 1 1 1];
      force_feedback_input = emg_value/12;
      state stim_n
        entry: user_output = 3005;
        return_force = 6;
        state stim_on
          during:
          pulsewidth = func.commonElectrode_4ch_stim(th_max,th_min,def_current,-def_current/4,0,'n','pw');
          current = func.commonElectrode_4ch_stim(th_max,th_min,def_current,-def_current/4,0,'n','cr');
          stim_status = func.commonElectrode_4ch_stim(th_max,th_min,def_current,-def_current/4,0,'n','lg');
          %ch3
        state stim_off [commented out]
          during:
          pulsewidth = func.commonElectrode_4ch_stim([0 0 0 0],th_min,def_current,-def_current/4,0,'e','pw');
          current = func.commonElectrode_4ch_stim([0 0 0 0],th_min,def_current,-def_current/4,0,'e','cr');
          %ch3
        (default) -> freeform_chart.force_feedback.stim_n.stim_on
        freeform_chart.force_feedback.stim_n.stim_on -> freeform_chart.force_feedback.stim_n.stim_off [commented out] : after(input_freq,sec)
        freeform_chart.force_feedback.stim_n.stim_off -> freeform_chart.force_feedback.stim_n.stim_on [commented out] : after(input_freq,sec)
      state pos_nw6
        entry: user_output = 3004;
        return_force = 4.5;
        state stim_on
          during:
          pulsewidth = func.commonElectrode_4ch_stim(th_max,th_min,def_current,-def_current/4,0,'nw','pw');
          current = func.commonElectrode_4ch_stim(th_max,th_min,def_current,-def_current/4,0,'nw','cr');
          stim_status = func.commonElectrode_4ch_stim(th_max,th_min,def_current,-def_current/4,0,'nw','lg');
          %ch3
        state stim_off
          during:
          pulsewidth = func.commonElectrode_4ch_stim(stim_off_pw,th_min,def_current,-def_current/4,0,'nw','pw');
          current = func.commonElectrode_4ch_stim(stim_off_pw,th_min,def_current,-def_current/4,0,'nw','cr');
          stim_status = func.commonElectrode_4ch_stim(stim_off_pw,th_min,def_current,-def_current/4,0,'nw','lg');
          %ch3
        (default) -> freeform_chart.force_feedback.pos_nw6.stim_on
        freeform_chart.force_feedback.pos_nw6.stim_on -> freeform_chart.force_feedback.pos_nw6.stim_off : after(0.2,sec)
        freeform_chart.force_feedback.pos_nw6.stim_off -> freeform_chart.force_feedback.pos_nw6.stim_on : after(0.2,sec)
      state pos_nw9
        entry: user_output = 3006;
        return_force = 7.5;
        state stim_on
          during:
          pulsewidth = func.commonElectrode_4ch_stim(th_max,th_min,def_current,-def_current/4,0,'ne','pw');
          current = func.commonElectrode_4ch_stim(th_max,th_min,def_current,-def_current/4,0,'ne','cr');
          stim_status = func.commonElectrode_4ch_stim(th_max,th_min,def_current,-def_current/4,0,'ne','lg');
          %ch3
        state stim_off
          during:
          pulsewidth = func.commonElectrode_4ch_stim(stim_off_pw,th_min,def_current,-def_current/4,0,'ne','pw');
          current = func.commonElectrode_4ch_stim(stim_off_pw,th_min,def_current,-def_current/4,0,'ne','cr');
          stim_status = func.commonElectrode_4ch_stim(stim_off_pw,th_min,def_current,-def_current/4,0,'ne','lg');
          %ch3
        (default) -> freeform_chart.force_feedback.pos_nw9.stim_on
        freeform_chart.force_feedback.pos_nw9.stim_on -> freeform_chart.force_feedback.pos_nw9.stim_off : after(0.2,sec)
        freeform_chart.force_feedback.pos_nw9.stim_off -> freeform_chart.force_feedback.pos_nw9.stim_on : after(0.2,sec)
      state pos_nw10
        entry: user_output = 3007;
        return_force = 9;
        state stim_on
          during:
          pulsewidth = func.commonElectrode_4ch_stim(th_max,th_min,def_current,-def_current/4,0,'e','pw');
          current = func.commonElectrode_4ch_stim(th_max,th_min,def_current,-def_current/4,0,'e','cr');
          stim_status = func.commonElectrode_4ch_stim(th_max,th_min,def_current,-def_current/4,0,'e','lg');
          %ch3
        state stim_off [commented out]
          during:
          pulsewidth = func.commonElectrode_4ch_stim(stim_off_pw,th_min,def_current,-def_current/4,0,'e','pw');
          current = func.commonElectrode_4ch_stim(stim_off_pw,th_min,def_current,-def_current/4,0,'e','cr');
          stim_status = func.commonElectrode_4ch_stim(stim_off_pw,th_min,def_current,-def_current/4,0,'e','lg');
          %ch3
        (default) -> freeform_chart.force_feedback.pos_nw10.stim_on
        freeform_chart.force_feedback.pos_nw10.stim_on -> freeform_chart.force_feedback.pos_nw10.stim_off [commented out] : after(0.2,sec)
        freeform_chart.force_feedback.pos_nw10.stim_off -> freeform_chart.force_feedback.pos_nw10.stim_on [commented out] : after(0.2,sec)
      state forcefeedback_3
        entry: user_output = 3003;
        return_force = 3;
        state stim_on
          during:
          pulsewidth = func.commonElectrode_4ch_stim(th_max,th_min,def_current,-def_current/4,0,'w','pw');
          current = func.commonElectrode_4ch_stim(th_max,th_min,def_current,-def_current/4,0,'w','cr');
          stim_status = func.commonElectrode_4ch_stim(th_max,th_min,def_current,-def_current/4,0,'w','lg');
          %ch3
        state stim_off [commented out]
          during:
          pulsewidth = func.commonElectrode_4ch_stim(stim_off_pw,th_min,def_current,-def_current/4,0,'nw','pw');
          current = func.commonElectrode_4ch_stim(stim_off_pw,th_min,def_current,-def_current/4,0,'nw','cr');
          stim_status = func.commonElectrode_4ch_stim(stim_off_pw,th_min,def_current,-def_current/4,0,'nw','lg');
          %ch3
        (default) -> freeform_chart.force_feedback.forcefeedback_3.stim_on
        freeform_chart.force_feedback.forcefeedback_3.stim_on -> freeform_chart.force_feedback.forcefeedback_3.stim_off [commented out] : after(0.2,sec)
        freeform_chart.force_feedback.forcefeedback_3.stim_off -> freeform_chart.force_feedback.forcefeedback_3.stim_on [commented out] : after(0.2,sec)
      state forcefeedback_2
        entry: user_output = 3002;
        return_force = 1.5;
        state stim_on
          during:
          pulsewidth = func.commonElectrode_4ch_stim(th_max,th_min,def_current,-def_current/4,0,'w','pw');
          current = func.commonElectrode_4ch_stim(th_max,th_min,def_current,-def_current/4,0,'w','cr');
          stim_status = func.commonElectrode_4ch_stim(th_max,th_min,def_current,-def_current/4,0,'w','lg');
          %ch3
        state stim_off
          during:
          pulsewidth = func.commonElectrode_4ch_stim(stim_off_pw,th_min,def_current,-def_current/4,0,'w','pw');
          current = func.commonElectrode_4ch_stim(stim_off_pw,th_min,def_current,-def_current/4,0,'w','cr');
          stim_status = func.commonElectrode_4ch_stim(stim_off_pw,th_min,def_current,-def_current/4,0,'w','lg');
          %ch3
        (default) -> freeform_chart.force_feedback.forcefeedback_2.stim_on
        freeform_chart.force_feedback.forcefeedback_2.stim_on -> freeform_chart.force_feedback.forcefeedback_2.stim_off : after(0.2,sec)
        freeform_chart.force_feedback.forcefeedback_2.stim_off -> freeform_chart.force_feedback.forcefeedback_2.stim_on : after(0.2,sec)
      state pos_nw11
        entry: user_output = 3008;
        return_force = 10.5;
        state stim_on
          during:
          pulsewidth = func.commonElectrode_4ch_stim(th_max,th_min,def_current,-def_current/4,0,'e','pw');
          current = func.commonElectrode_4ch_stim(th_max,th_min,def_current,-def_current/4,0,'e','cr');
          stim_status = func.commonElectrode_4ch_stim(th_max,th_min,def_current,-def_current/4,0,'e','lg');
          %ch3
        state stim_off
          during:
          pulsewidth = func.commonElectrode_4ch_stim(stim_off_pw,th_min,def_current,-def_current/4,0,'e','pw');
          current = func.commonElectrode_4ch_stim(stim_off_pw,th_min,def_current,-def_current/4,0,'e','cr');
          stim_status = func.commonElectrode_4ch_stim(stim_off_pw,th_min,def_current,-def_current/4,0,'e','lg');
          %ch3
        (default) -> freeform_chart.force_feedback.pos_nw11.stim_on
        freeform_chart.force_feedback.pos_nw11.stim_on -> freeform_chart.force_feedback.pos_nw11.stim_off : after(0.2,sec)
        freeform_chart.force_feedback.pos_nw11.stim_off -> freeform_chart.force_feedback.pos_nw11.stim_on : after(0.2,sec)
      state stim_w
        entry: user_output = 3001;
        return_force = 0;
        state stim_on
          during:
          pulsewidth = func.commonElectrode_4ch_stim(th_max,th_min,def_current,-def_current/4,0,'sw','pw');
          current = func.commonElectrode_4ch_stim(th_max,th_min,def_current,-def_current/4,0,'sw','cr');
          stim_status = func.commonElectrode_4ch_stim(th_max,th_min,def_current,-def_current/4,0,'sw','lg');
          %ch3
        state stim_off
          during:
          pulsewidth = func.commonElectrode_4ch_stim(stim_off_pw,th_min,def_current,-def_current/4,0,'sw','pw');
          current = func.commonElectrode_4ch_stim(stim_off_pw,th_min,def_current,-def_current/4,0,'sw','cr');
          stim_status = func.commonElectrode_4ch_stim(stim_off_pw,th_min,def_current,-def_current/4,0,'sw','lg');
          %ch3
        (default) -> freeform_chart.force_feedback.stim_w.stim_on
        freeform_chart.force_feedback.stim_w.stim_on -> freeform_chart.force_feedback.stim_w.stim_off : after(0.2,sec)
        freeform_chart.force_feedback.stim_w.stim_off -> freeform_chart.force_feedback.stim_w.stim_on : after(0.2,sec)
      state stim_e
        entry: user_output = 3009;
        return_force = 12;
        state stim_on
          during:
          pulsewidth = func.commonElectrode_4ch_stim(th_max,th_min,def_current,-def_current/4,0,'se','pw');
          current = func.commonElectrode_4ch_stim(th_max,th_min,def_current,-def_current/4,0,'se','cr');
          stim_status = func.commonElectrode_4ch_stim(th_max,th_min,def_current,-def_current/4,0,'se','lg');
          %ch3
        state stim_off
          during:
          pulsewidth = func.commonElectrode_4ch_stim(stim_off_pw,th_min,def_current,-def_current/4,0,'se','pw');
          current = func.commonElectrode_4ch_stim(stim_off_pw,th_min,def_current,-def_current/4,0,'se','cr');
          stim_status = func.commonElectrode_4ch_stim(stim_off_pw,th_min,def_current,-def_current/4,0,'se','lg');
          %ch3
        (default) -> freeform_chart.force_feedback.stim_e.stim_on
        freeform_chart.force_feedback.stim_e.stim_on -> freeform_chart.force_feedback.stim_e.stim_off : after(0.2,sec)
        freeform_chart.force_feedback.stim_e.stim_off -> freeform_chart.force_feedback.stim_e.stim_on : after(0.2,sec)
      (default) -> freeform_chart.force_feedback.stim_n
      freeform_chart.force_feedback.pos_nw9 -> freeform_chart.force_feedback.stim_n [order 1] : [force_feedback_input <= 0.5625]
      freeform_chart.force_feedback.stim_n -> freeform_chart.force_feedback.pos_nw9 [order 2] : [force_feedback_input > 0.5625]
      freeform_chart.force_feedback.stim_n -> freeform_chart.force_feedback.pos_nw6 [order 1] : [force_feedback_input <= 0.4375]
      freeform_chart.force_feedback.pos_nw6 -> freeform_chart.force_feedback.stim_n [order 2] : [force_feedback_input > 0.4375]
      freeform_chart.force_feedback.pos_nw6 -> freeform_chart.force_feedback.forcefeedback_3 [order 1] : [force_feedback_input <= 0.3125]
      freeform_chart.force_feedback.forcefeedback_3 -> freeform_chart.force_feedback.pos_nw6 [order 2] : [force_feedback_input > 0.3125]
      freeform_chart.force_feedback.pos_nw9 -> freeform_chart.force_feedback.pos_nw10 [order 2] : [force_feedback_input > 0.6875]
      freeform_chart.force_feedback.pos_nw10 -> freeform_chart.force_feedback.pos_nw9 [order 1] : [force_feedback_input <= 0.6875]
      freeform_chart.force_feedback.pos_nw10 -> freeform_chart.force_feedback.pos_nw11 [order 2] : [force_feedback_input > 0.8125]
      freeform_chart.force_feedback.forcefeedback_3 -> freeform_chart.force_feedback.forcefeedback_2 [order 1] : [force_feedback_input <= 0.1875]
      freeform_chart.force_feedback.forcefeedback_2 -> freeform_chart.force_feedback.forcefeedback_3 [order 1] : [force_feedback_input > 0.1875]
      freeform_chart.force_feedback.pos_nw11 -> freeform_chart.force_feedback.pos_nw10 [order 1] : [force_feedback_input <= 0.8125]
      freeform_chart.force_feedback.forcefeedback_2 -> freeform_chart.force_feedback.stim_w [order 2] : [force_feedback_input <= 0.0625]
      freeform_chart.force_feedback.stim_w -> freeform_chart.force_feedback.forcefeedback_2 : [force_feedback_input > 0.0625]
      freeform_chart.force_feedback.pos_nw11 -> freeform_chart.force_feedback.stim_e [order 2] : [force_feedback_input > 0.9375]
      freeform_chart.force_feedback.stim_e -> freeform_chart.force_feedback.pos_nw11 : [force_feedback_input <= 0.9375]
    state cont_pos
      entry:
      init_for_integrator = return_cont_pos;
    state wait3
      entry: pulsewidth = func.commonElectrode_4ch_emgstim([1 1 1 1],th_min,def_current,-def_current/4,0,'pw');
      current = func.commonElectrode_4ch_emgstim([1 1 1 1],th_min,def_current,-def_current/4,0,'cr');
      stim_status = func.commonElectrode_4ch_emgstim([1 1 1 1],th_min,def_current,-def_current/4,0,'lg');
    state wait5
    state disc_opcl
      entry:
      init_for_integrator = return_opcl;
    state stim_pos
      entry:
      reset_integrator = 0;
      init_for_integrator = return_cont_pos;
      during:
      pulsewidth = func.commonElectrode_4ch_pos(th_max, th_min, def_current, -def_current/4, 0, emg_value*30, 'pw');
      current = func.commonElectrode_4ch_pos(th_max, th_min, def_current, -def_current/4, 0, emg_value*30, 'cr');
      stim_status = func.commonElectrode_4ch_pos(th_max, th_min, def_current, -def_current/4, 0, emg_value*30, 'lg');
      user_output = emg_value*30;
      exit:
      return_cont_pos = emg_value;
    state wait1
      entry: pulsewidth = func.commonElectrode_4ch_emgstim([1 1 1 1],th_min,def_current,-def_current/4,0,'pw');
      current = func.commonElectrode_4ch_emgstim([1 1 1 1],th_min,def_current,-def_current/4,0,'cr');
      stim_status = func.commonElectrode_4ch_emgstim([1 1 1 1],th_min,def_current,-def_current/4,0,'lg');
    state wait6
    state hand_openclosed
      entry: reset_integrator = 0;
      during: stim_off_pw= [1 1 1 1]
      state neutral
        entry: user_output = 2001;
        return_opcl = 0;
        state pos_west2
          during:
          pulsewidth = func.commonElectrode_4ch_stim(stim_off_pw,th_min,def_current,-def_current/4,0,'ns','pw');
          current = func.commonElectrode_4ch_stim(stim_off_pw,th_min,def_current,-def_current/4,0,'ns','cr');
          stim_status = func.commonElectrode_4ch_stim(stim_off_pw,th_min,def_current,-def_current/4,0,'ns','lg');
          %ch3
      state level1
        entry: user_output = 2002;
        return_opcl = 4.5;
        state pos_west1
          during:
          pulsewidth = func.commonElectrode_4ch_stim(th_max,th_min,def_current,-def_current/4,0,'ns','pw');
          current = func.commonElectrode_4ch_stim(th_max,th_min,def_current,-def_current/4,0,'ns','cr');
          stim_status = func.commonElectrode_4ch_stim(th_max,th_min,def_current,-def_current/4,0,'ns','lg');
          %ch3
        state pos_west2
          during:
          pulsewidth = func.commonElectrode_4ch_stim(stim_off_pw,th_min,def_current,-def_current/4,0,'ns','pw');
          current = func.commonElectrode_4ch_stim(stim_off_pw,th_min,def_current,-def_current/4,0,'ns','cr');
          stim_status = func.commonElectrode_4ch_stim(stim_off_pw,th_min,def_current,-def_current/4,0,'ns','lg');
          %ch3
        (default) -> freeform_chart.hand_openclosed.level1.pos_west1
        freeform_chart.hand_openclosed.level1.pos_west1 -> freeform_chart.hand_openclosed.level1.pos_west2 : after(0.5,sec)
        freeform_chart.hand_openclosed.level1.pos_west2 -> freeform_chart.hand_openclosed.level1.pos_west1 : after(0.5,sec)
      state level2
        entry:  user_output = 2003;
        return_opcl = 7.5;
        state pos_west1
          during:
          pulsewidth = func.commonElectrode_4ch_stim(th_max,th_min,def_current,-def_current/4,0,'ns','pw');
          current = func.commonElectrode_4ch_stim(th_max,th_min,def_current,-def_current/4,0,'ns','cr');
          stim_status = func.commonElectrode_4ch_stim(th_max,th_min,def_current,-def_current/4,0,'ns','lg');
          %ch3
        state pos_west2
          during:
          pulsewidth = func.commonElectrode_4ch_stim(stim_off_pw,th_min,def_current,-def_current/4,0,'ns','pw');
          current = func.commonElectrode_4ch_stim(stim_off_pw,th_min,def_current,-def_current/4,0,'ns','cr');
          stim_status = func.commonElectrode_4ch_stim(stim_off_pw,th_min,def_current,-def_current/4,0,'ns','lg');
          %ch3
        (default) -> freeform_chart.hand_openclosed.level2.pos_west1
        freeform_chart.hand_openclosed.level2.pos_west1 -> freeform_chart.hand_openclosed.level2.pos_west2 : after(0.25,sec)
        freeform_chart.hand_openclosed.level2.pos_west2 -> freeform_chart.hand_openclosed.level2.pos_west1 : after(0.25,sec)
      state level3
        entry:  user_output = 2004;
        return_opcl = 12;
        state pos_west1
          during:
          pulsewidth = func.commonElectrode_4ch_stim(th_max,th_min,def_current,-def_current/4,0,'ns','pw');
          current = func.commonElectrode_4ch_stim(th_max,th_min,def_current,-def_current/4,0,'ns','cr');
          stim_status = func.commonElectrode_4ch_stim(th_max,th_min,def_current,-def_current/4,0,'ns','lg');
          %ch3
        (default) -> freeform_chart.hand_openclosed.level3.pos_west1
      (default) -> freeform_chart.hand_openclosed.neutral
      freeform_chart.hand_openclosed.neutral -> freeform_chart.hand_openclosed.level1 : [emg_value >= 3]
      freeform_chart.hand_openclosed.level1 -> freeform_chart.hand_openclosed.neutral [order 2] : [emg_value < 3]
      freeform_chart.hand_openclosed.level1 -> freeform_chart.hand_openclosed.level2 [order 1] : [emg_value >= 6]
      freeform_chart.hand_openclosed.level2 -> freeform_chart.hand_openclosed.level1 [order 2] : [emg_value < 6]
      freeform_chart.hand_openclosed.level2 -> freeform_chart.hand_openclosed.level3 [order 1] : [emg_value >= 9]
      freeform_chart.hand_openclosed.level3 -> freeform_chart.hand_openclosed.level2 : [emg_value < 9]
    (default) -> freeform_chart.stim_control
    wait -> wait4 : {reset_integrator = 1;}
    freeform_chart.hand_openclosed -> freeform_chart.stim_control : [stim_command ~= 2]
    freeform_chart.feedback_change_indicator4 -> disc_pos [order 1] : [jump_n == stim_command && stim_command == 1]
    disc_pos -> wait : after(0.25,sec)
    wait4 -> freeform_chart.handposition_map1 : after(0.25,sec)
    freeform_chart.handposition_map1 -> freeform_chart.stim_control : [stim_command ~= 1]
    freeform_chart.stim_pos -> freeform_chart.stim_control : [stim_command ~= 4]
    freeform_chart.force_feedback -> freeform_chart.stim_control : [stim_command ~= 3]
    disc_force -> wait2 : after(0.25,sec)
    wait2 -> wait7 : {reset_integrator = 1;}
    freeform_chart.stim_control -> freeform_chart.feedback_change_indicator4 : after(0.5,sec)[stim_command ~= 0]
    freeform_chart.feedback_change_indicator4 -> cont_pos [order 4] : [jump_n == stim_command && stim_command == 4]
    freeform_chart.feedback_change_indicator4 -> disc_force [order 3] : [jump_n == stim_command && stim_command == 3]
    wait7 -> freeform_chart.force_feedback : after(0.25,sec)
    cont_pos -> wait3 : after(0.25,sec)
    wait3 -> wait5 : {reset_integrator = 1;}
    freeform_chart.feedback_change_indicator4 -> disc_opcl [order 2] : [jump_n == stim_command && stim_command == 2]
    wait5 -> freeform_chart.stim_pos : after(0.25,sec)
    disc_opcl -> wait1 : after(0.25,sec)
    wait1 -> wait6 : {reset_integrator = 1;}
    wait6 -> freeform_chart.hand_openclosed : after(0.25,sec)
  (default) -> init
  threshold_val_min_ch1 -> threshold_val_max_ch1 : [n == 2]
  init -> threshold_val_min_ch1 : [n == 1]
  threshold_val_max_ch1 -> threshold_val_min_ch2 : [n == 3]
  threshold_val_min_ch2 -> threshold_val_max_ch2 : [n == 4]
  threshold_val_max_ch2 -> threshold_val_min_ch3 : [n ==5]
  threshold_val_min_ch3 -> threshold_val_max_ch3 : [n == 6]
  threshold_val_max_ch3 -> threshold_val_min_ch4 : [n == 7]
  threshold_val_max_ch4 -> stimfor_emg_thresholds : [n == 9]
  threshold_val_min_ch4 -> threshold_val_max_ch4 : [n == 8]
  selection -> preview [order 1] : [preview == 1]
  preview -> selection : [preview == 0]
  selection -> testbench [order 3] : [testbench == 1]
  stop2 -> selection
  testbench -> selection : [testbench == 0]
  selection -> freeform_chart [order 2] : [freeform == 1]
  freeform_chart -> selection : [freeform == 0]
  data: stimpw function_input; stimcr function_input; balancecr function_input; pausepw function_input; select_channel function_input; select_output function_input; output function_output; threshold_max function_input; threshold_min function_input; stimcr function_input; balancecr function_input; pausepw function_input; select_direction function_input; select_output function_input; output function_output; threshold_max function_input; threshold_min function_input; stimcr function_input; balancecr function_input; pausepw function_input; degree function_input; select_output function_input; output function_output; threshold_max function_input; threshold_min function_input; stimcr function_input; balancecr function_input; pausepw function_input; select_output function_input; output function_output; threshold_max function_input; threshold_min function_input; stimcr function_input; balancecr function_input; pausepw function_input; input_emg function_input; integrator_max function_input; select_output function_input; output function_output; threshold_max function_input; threshold_min function_input; stimcr function_input; balancecr function_input; pausepw function_input; force_feedback_value function_input; integrator_max function_input; select_output function_input; output function_output; th_max input size=[1 4]; th_min input size=[1 4]; n input; value_pw input; def_current input; single_click input; current output; pulsewidth output; stim_command input; swytch local; stim_status output; stim_off_pw local; reset_integrator output; jump_n local; c input; emg_value input; force_feedback_input local; user_output output; preview_again input; preview input; freeform input; testbench input; init_for_integrator output; return_cont_pos local; return_pos local; return_force local; return_opcl local; test_command input; test_value input; test_output output; test_force_feedback_input local; ready_for_stim output
  function output = commonElectrode_4ch_threshold(stimpw,stimcr,balancecr,pausepw,select_channel,select_output):
    | function output = commonElectrode_4ch_threshold(stimpw,stimcr,balancecr,pausepw,select_channel,select_output)
    | % error checking
    | if(sign(stimcr) == sign(balancecr))
    |    error('Stimulation is not charge balanced'); 
    | end
    | % create single channel current vectors
    | ch1_cr = zeros(1,4)';
    | ch2_cr = zeros(1,4)';
    | ch3_cr = zeros(1,4)';
    | ch4_cr = zeros(1,4)';
    | % assign channel value to first element of each vector
    | ch1_cr(1) = 1; ch2_cr(1)=2; ch3_cr(1)= 3; ch4_cr(1)=4;
    | % assign stimcr,balancecr and pausecr(=0) to every current vector
    | ch1_cr(2) = stimcr; ch2_cr(2) = stimcr; ch3_cr(2) = stimcr; ch4_cr(2) = stimcr;
    | ch1_cr(3) = balancecr; ch2_cr(3) = balancecr; ch3_cr(3) = balancecr; ch4_cr(3) = balancecr;
    | ch1_cr(4) = 0; ch2_cr(4) = 0; ch3_cr(4) = 0; ch4_cr(4) = 0;
    | % -------current vectors completed-------
    | 
    | % create single channel pulsewidth vectors
    | ch1_pw = zeros(1,4)';
    | ch2_pw = zeros(1,4)';
    | ch3_pw = zeros(1,4)';
    | ch4_pw = zeros(1,4)';
    | % assign channel value to first element of each vectors
    | ch1_pw(1) = 1; ch2_pw(1) = 2; ch3_pw(1) = 3; ch4_pw(1) = 4;
    | % assign stimpw to every pulsewidth vector
    | ch1_pw(2) = stimpw; ch2_pw(2) = stimpw; ch3_pw(2) = stimpw; ch4_pw(2) = stimpw;
    | % calculate total charge to balance for each channel
    | c2b_ch1 = abs(ch1_pw(2)*stimcr);
    | c2b_ch2 = abs(ch2_pw(2)*stimcr);
    | c2b_ch3 = abs(ch3_pw(2)*stimcr);
    | c2b_ch4 = abs(ch4_pw(2)*stimcr);
    | % calculate and assign balancepw
    | ch1_pw(3) = c2b_ch1/abs(balancecr);
    | ch2_pw(3) = c2b_ch2/abs(balancecr);
    | ch3_pw(3) = c2b_ch3/abs(balancecr);
    | ch4_pw(3) = c2b_ch4/abs(balancecr);
    | % assign pausepw
    | ch1_pw(4) = pausepw; ch2_pw(4) = pausepw; ch3_pw(4) = pausepw; ch4_pw(4) = pausepw;
    | % create null vectors for current and pulsewidth
    | null_ch1 = zeros(1,4)'; null_ch1(1) = 1;
    | null_ch2 = zeros(1,4)'; null_ch2(1) = 2;
    | null_ch3 = zeros(1,4)'; null_ch3(1) = 3;
    | null_ch4 = zeros(1,4)'; null_ch4(1) = 4;
    | 
    | % create output matrices depending on select_channel and select_output
    | if(select_channel == 1 && strcmp('pw',select_output))
    |    output = [ch1_pw, null_ch2, null_ch3, null_ch4];
    | elseif (select_channel == 2 && strcmp('pw',select_output))
    |    output = [null_ch1, ch2_pw, null_ch3, null_ch4];
    | elseif (select_channel == 3 && strcmp('pw',select_output))
    |    output = [null_ch1, null_ch2, ch3_pw, null_ch4];
    | elseif (select_channel == 4 && strcmp('pw',select_output))
    |    output = [null_ch1, null_ch2, null_ch3, ch4_pw];     
    | elseif (select_channel == 1 && strcmp('cr',select_output))
    |    output = [ch1_cr, null_ch2, null_ch3, null_ch4];
    | elseif (select_channel == 2 && strcmp('cr',select_output))
    |    output = [null_ch1, ch2_cr, null_ch3, null_ch4];
    | elseif (select_channel == 3 && strcmp('cr',select_output))
    |    output = [null_ch1, null_ch2, ch3_cr, null_ch4];
    | elseif (select_channel == 4 && strcmp('cr',select_output))
    |    output = [null_ch1, null_ch2, null_ch3, ch4_cr];
    | elseif (stimpw == 0 && strcmp('lg',select_output))
    |    output = 0;
    | elseif (stimpw ~= 0 && strcmp('lg',select_output))
    |    output = 1;
    | else
    |     error('Function paramater error, check parameters for spelling, etc.');    
    | end
  function output = commonElectrode_4ch_stim(threshold_max,threshold_min,stimcr,balancecr,pausepw,select_direction,select_output):
    | function output = commonElectrode_4ch_stim(threshold_max,threshold_min,stimcr,balancecr,pausepw,select_direction,select_output)
    | % create single channel current vectors
    | ch1_cr = zeros(1,4)';
    | ch2_cr = zeros(1,4)';
    | ch3_cr = zeros(1,4)';
    | ch4_cr = zeros(1,4)';
    | % assign channel value to first element of each vector
    | ch1_cr(1) = 1; ch2_cr(1)=2; ch3_cr(1)= 3; ch4_cr(1)=4;
    | % assign stimcr,balancecr and pausecr(=0) to every current vector
    | ch1_cr(2) = stimcr; ch2_cr(2) = stimcr; ch3_cr(2) = stimcr; ch4_cr(2) = stimcr;
    | ch1_cr(3) = balancecr; ch2_cr(3) = balancecr; ch3_cr(3) = balancecr; ch4_cr(3) = balancecr;
    | ch1_cr(4) = 0; ch2_cr(4) = 0; ch3_cr(4) = 0; ch4_cr(4) = 0;
    | % -------current vectors completed-------
    | 
    | % create single channel pulsewidth vectors
    | ch1_pw = zeros(1,4)';
    | ch2_pw = zeros(1,4)';
    | ch3_pw = zeros(1,4)';
    | ch4_pw = zeros(1,4)';
    | % assign channel value to first element of each vectors
    | ch1_pw(1) = 1; ch2_pw(1) = 2; ch3_pw(1) = 3; ch4_pw(1) = 4;
    | % assign threshold values to every pulsewidth vector
    | ch1_pw(2) = threshold_max(1); ch2_pw(2) = threshold_max(2); ch3_pw(2) = threshold_max(3); ch4_pw(2) = threshold_max(4);
    | % calculate total charge to balance for each channel
    | c2b_ch1 = abs(ch1_pw(2)*stimcr);
    | c2b_ch2 = abs(ch2_pw(2)*stimcr);
    | c2b_ch3 = abs(ch3_pw(2)*stimcr);
    | c2b_ch4 = abs(ch4_pw(2)*stimcr);
    | % calculate and assign balancepw
    | ch1_pw(3) = c2b_ch1/abs(balancecr);
    | ch2_pw(3) = c2b_ch2/abs(balancecr);
    | ch3_pw(3) = c2b_ch3/abs(balancecr);
    | ch4_pw(3) = c2b_ch4/abs(balancecr);
    | % assign pausepw
    | ch1_pw(4) = pausepw; ch2_pw(4) = pausepw; ch3_pw(4) = pausepw; ch4_pw(4) = pausepw;
    | % create null vectors for current and pulsewidth
    | null_ch1 = zeros(1,4)'; null_ch1(1) = 1;
    | null_ch2 = zeros(1,4)'; null_ch2(1) = 2;
    | null_ch3 = zeros(1,4)'; null_ch3(1) = 3;
    | null_ch4 = zeros(1,4)'; null_ch4(1) = 4;
    | % create output matrices depending on select_channel and select_output
    | if(strcmp('n',select_direction) && strcmp('pw',select_output))
    |    output = [ch1_pw, null_ch2, null_ch3, null_ch4];
    | elseif (strcmp('s',select_direction) && strcmp('pw',select_output))
    |    output = [null_ch1, ch2_pw, null_ch3, null_ch4];
    | elseif (strcmp('w',select_direction) && strcmp('pw',select_output))
    |    output = [null_ch1, null_ch2, ch3_pw, null_ch4];
    | elseif (strcmp('e',select_direction) && strcmp('pw',select_output))
    |    output = [null_ch1, null_ch2, null_ch3, ch4_pw];     
    | elseif (strcmp('nw',select_direction) && strcmp('pw',select_output))
    |    output = [ch1_pw, null_ch2, ch3_pw, null_ch4];
    | elseif (strcmp('ne',select_direction) && strcmp('pw',select_output))
    |    output = [ch1_pw, null_ch2, null_ch3, ch4_pw];
    | elseif (strcmp('sw',select_direction) && strcmp('pw',select_output))
    |    output = [null_ch1, ch2_pw, ch3_pw, null_ch4];
    | elseif (strcmp('se',select_direction) && strcmp('pw',select_output))
    |    output = [null_ch1, ch2_pw, null_ch3, ch4_pw];   
    | elseif(strcmp('n',select_direction) && strcmp('cr',select_output))
    |    output = [ch1_cr, null_ch2, null_ch3, null_ch4];
    | elseif (strcmp('s',select_direction) && strcmp('cr',select_output))
    |    output = [null_ch1, ch2_cr, null_ch3, null_ch4];
    | elseif (strcmp('w',select_direction) && strcmp('cr',select_output))
    |    output = [null_ch1, null_ch2, ch3_cr, null_ch4];
    | elseif (strcmp('e',select_direction) && strcmp('cr',select_output))
    |    output = [null_ch1, null_ch2, null_ch3, ch4_cr];     
    | elseif (strcmp('nw',select_direction) && strcmp('cr',select_output))
    |    output = [ch1_cr, null_ch2, ch3_cr, null_ch4];
    | elseif (strcmp('ne',select_direction) && strcmp('cr',select_output))
    |    output = [ch1_cr, null_ch2, null_ch3, ch4_cr];
    | elseif (strcmp('sw',select_direction) && strcmp('cr',select_output))
    |    output = [null_ch1, ch2_cr, ch3_cr, null_ch4];
    | elseif (strcmp('se',select_direction) && strcmp('cr',select_output))
    |    output = [null_ch1, ch2_cr, null_ch3, ch4_cr];
    | % unconventional directions
    | elseif(strcmp('ns',select_direction) && strcmp('pw',select_output))
    |    output = [ch1_pw, ch2_pw, null_ch3, null_ch4];
    | elseif (strcmp('we',select_direction) && strcmp('pw',select_output))
    |    output = [null_ch1, null_ch2, ch3_pw, ch4_pw];
    | elseif(strcmp('ns',select_direction) && strcmp('cr',select_output))
    |    output = [ch1_cr, ch2_cr, null_ch3, null_ch4];
    | elseif (strcmp('we',select_direction) && strcmp('cr',select_output))
    |    output = [null_ch1, null_ch2, ch3_cr, ch4_cr];
    | elseif (int8(all(eq(threshold_max,zeros(1,4)))) && strcmp('lg',select_output))
    |    output = 0;
    | elseif (int8(~all(eq(threshold_max,zeros(1,4)))) && strcmp('lg',select_output))
    |    output = 1;
    | else
    |     error('Function paramater error, check parameters for spelling, etc.');    
    | end
    | end
  function output = commonElectrode_4ch_pos(threshold_max,threshold_min,stimcr,balancecr,pausepw,degree,select_output):
    | function output = commonElectrode_4ch_pos(threshold_max,threshold_min,stimcr,balancecr,pausepw,degree,select_output)
    | % create single channel current vectors
    | ch1_cr = zeros(1,4)';
    | ch2_cr = zeros(1,4)';
    | ch3_cr = zeros(1,4)';
    | ch4_cr = zeros(1,4)';
    | % assign channel value to first element of each vector
    | ch1_cr(1) = 1; ch2_cr(1)=2; ch3_cr(1)= 3; ch4_cr(1)=4;
    | % assign stimcr,balancecr and pausecr(=0) to every current vector
    | ch1_cr(2) = stimcr; ch2_cr(2) = stimcr; ch3_cr(2) = stimcr; ch4_cr(2) = stimcr;
    | ch1_cr(3) = balancecr; ch2_cr(3) = balancecr; ch3_cr(3) = balancecr; ch4_cr(3) = balancecr;
    | ch1_cr(4) = 0; ch2_cr(4) = 0; ch3_cr(4) = 0; ch4_cr(4) = 0;
    | % -------current vectors completed-------
    | 
    | % create single channel pulsewidth vectors
    | ch1_pw = zeros(1,4)';
    | ch2_pw = zeros(1,4)';
    | ch3_pw = zeros(1,4)';
    | ch4_pw = zeros(1,4)';
    | % assign channel value to first element of each vectors
    | ch1_pw(1) = 1; ch2_pw(1) = 2; ch3_pw(1) = 3; ch4_pw(1) = 4;
    | 
    | % linear map from 0 to 359
    | % calculate the slope for each segment of 90 degrees
    | slope_ch1 = threshold_max(1)/90;
    | slope_ch2 = threshold_max(2)/90;
    | slope_ch3 = threshold_max(3)/90;
    | slope_ch4 = threshold_max(4)/90;
    | 
    | if (0 <= degree) && (degree < 90)
    |     ch1_pw(2) = threshold_max(1) - slope_ch1*degree;
    |     ch3_pw(2) = slope_ch3*degree;
    |     ch2_pw(2) = 0;
    |     ch4_pw(2) = 0;
    | elseif (90 <= degree) && (degree < 180)
    |     deg_m90 = degree - 90;
    |     ch1_pw(2) = 0;
    |     ch3_pw(2) = threshold_max(3) - slope_ch3*deg_m90;
    |     ch2_pw(2) = slope_ch2*deg_m90;
    |     ch4_pw(2) = 0;
    | elseif (180 <= degree) && (degree < 270)
    |     deg_m180 = degree - 180;
    |     ch1_pw(2) = 0;
    |     ch3_pw(2) = 0;
    |     ch2_pw(2) = threshold_max(2) - slope_ch2*deg_m180;
    |     ch4_pw(2) = slope_ch4*deg_m180;
    | elseif (270 <= degree) && (degree < 361)
    |     deg_m270 = degree - 270;
    |     ch1_pw(2) = slope_ch1*deg_m270;
    |     ch3_pw(2) = 0;
    |     ch2_pw(2) = 0;
    |     ch4_pw(2) = threshold_max(4) - slope_ch4*deg_m270;
    | end
    | 
    | % calculate total charge to balance for each channel
    | c2b_ch1 = abs(ch1_pw(2)*stimcr);
    | c2b_ch2 = abs(ch2_pw(2)*stimcr);
    | c2b_ch3 = abs(ch3_pw(2)*stimcr);
    | c2b_ch4 = abs(ch4_pw(2)*stimcr);
    | % calculate and assign balancepw
    | ch1_pw(3) = c2b_ch1/abs(balancecr);
    | ch2_pw(3) = c2b_ch2/abs(balancecr);
    | ch3_pw(3) = c2b_ch3/abs(balancecr);
    | ch4_pw(3) = c2b_ch4/abs(balancecr);
    | % assign pausepw
    | ch1_pw(4) = pausepw; ch2_pw(4) = pausepw; ch3_pw(4) = pausepw; ch4_pw(4) = pausepw;
    | % create null vectors for current and pulsewidth
    | null_ch1 = zeros(1,4)'; null_ch1(1) = 1;
    | null_ch2 = zeros(1,4)'; null_ch2(1) = 2;
    | null_ch3 = zeros(1,4)'; null_ch3(1) = 3;
    | null_ch4 = zeros(1,4)'; null_ch4(1) = 4;
    | 
    | % create output matrices depending on select_channel and select_output
    | if(strcmp('pw',select_output))
    |    output = [ch1_pw, ch2_pw, ch3_pw, ch4_pw];
    | elseif(strcmp('cr',select_output))
    |    output = [ch1_cr, ch2_cr, ch3_cr, ch4_cr];
    | elseif (int8(all(eq(threshold_max,zeros(1,4)))) && strcmp('lg',select_output))
    |    output = 0;
    | elseif (int8(~all(eq(threshold_max,zeros(1,4)))) && strcmp('lg',select_output))
    |    output = 1;
    | else
    |     error('Function paramater error, check parameters for spelling, etc.');    
    | end
    | end
  function output = commonElectrode_4ch_emgstim(threshold_max,threshold_min,stimcr,balancecr,pausepw,select_output):
    | function output = commonElectrode_4ch_emgstim(threshold_max,threshold_min,stimcr,balancecr,pausepw,select_output)
    | % create single channel current vectors
    | ch1_cr = zeros(1,4)';
    | ch2_cr = zeros(1,4)';
    | ch3_cr = zeros(1,4)';
    | ch4_cr = zeros(1,4)';
    | % assign channel value to first element of each vector
    | ch1_cr(1) = 1; ch2_cr(1)=2; ch3_cr(1)= 3; ch4_cr(1)=4;
    | % assign stimcr,balancecr and pausecr(=0) to every current vector
    | ch1_cr(2) = stimcr; ch2_cr(2) = stimcr; ch3_cr(2) = stimcr; ch4_cr(2) = stimcr;
    | ch1_cr(3) = balancecr; ch2_cr(3) = balancecr; ch3_cr(3) = balancecr; ch4_cr(3) = balancecr;
    | ch1_cr(4) = 0; ch2_cr(4) = 0; ch3_cr(4) = 0; ch4_cr(4) = 0;
    | % -------current vectors completed-------
    | 
    | % create single channel pulsewidth vectors
    | ch1_pw = zeros(1,4)';
    | ch2_pw = zeros(1,4)';
    | ch3_pw = zeros(1,4)';
    | ch4_pw = zeros(1,4)';
    | % assign channel value to first element of each vectors
    | ch1_pw(1) = 1; ch2_pw(1) = 2; ch3_pw(1) = 3; ch4_pw(1) = 4;
    | % assign threshold values to every pulsewidth vector
    | ch1_pw(2) = threshold_max(1); ch2_pw(2) = threshold_max(2); ch3_pw(2) = threshold_max(3); ch4_pw(2) = threshold_max(4);
    | % calculate total charge to balance for each channel
    | c2b_ch1 = abs(ch1_pw(2)*stimcr);
    | c2b_ch2 = abs(ch2_pw(2)*stimcr);
    | c2b_ch3 = abs(ch3_pw(2)*stimcr);
    | c2b_ch4 = abs(ch4_pw(2)*stimcr);
    | % calculate and assign balancepw
    | ch1_pw(3) = c2b_ch1/abs(balancecr);
    | ch2_pw(3) = c2b_ch2/abs(balancecr);
    | ch3_pw(3) = c2b_ch3/abs(balancecr);
    | ch4_pw(3) = c2b_ch4/abs(balancecr);
    | % assign pausepw
    | ch1_pw(4) = pausepw; ch2_pw(4) = pausepw; ch3_pw(4) = pausepw; ch4_pw(4) = pausepw;
    | % create null vectors for current and pulsewidth
    | null_ch1 = zeros(1,4)'; null_ch1(1) = 1;
    | null_ch2 = zeros(1,4)'; null_ch2(1) = 2;
    | null_ch3 = zeros(1,4)'; null_ch3(1) = 3;
    | null_ch4 = zeros(1,4)'; null_ch4(1) = 4;
    | % create output matrices depending on select_channel and select_output
    | if(strcmp('pw',select_output))
    |    output = [ch1_pw, ch2_pw, ch3_pw, ch4_pw];  
    | elseif(strcmp('cr',select_output))
    |    output = [ch1_cr, ch2_cr, ch3_cr, ch4_cr];
    | elseif (int8(all(eq(threshold_max,zeros(1,4)))) && strcmp('lg',select_output))
    |    output = 0;
    | elseif (int8(~all(eq(threshold_max,zeros(1,4)))) && strcmp('lg',select_output))
    |    output = 1;
    | else
    |     error('Function paramater error, check parameters for spelling, etc.');    
    | end
    | end
  function output = commonElectrode_4ch_opcl(threshold_max,threshold_min,stimcr,balancecr,pausepw,input_emg,integrator_max,select_output):
    | function output = commonElectrode_4ch_opcl(threshold_max,threshold_min,stimcr,balancecr,pausepw,input_emg,integrator_max,select_output)
    | % create single channel current vectors
    | ch1_cr = zeros(1,4)';
    | ch2_cr = zeros(1,4)';
    | ch3_cr = zeros(1,4)';
    | ch4_cr = zeros(1,4)';
    | % assign channel value to first element of each vector
    | ch1_cr(1) = 1; ch2_cr(1)=2; ch3_cr(1)= 3; ch4_cr(1)=4;
    | % assign stimcr,balancecr and pausecr(=0) to every current vector
    | ch1_cr(2) = stimcr; ch2_cr(2) = stimcr; ch3_cr(2) = stimcr; ch4_cr(2) = stimcr;
    | ch1_cr(3) = balancecr; ch2_cr(3) = balancecr; ch3_cr(3) = balancecr; ch4_cr(3) = balancecr;
    | ch1_cr(4) = 0; ch2_cr(4) = 0; ch3_cr(4) = 0; ch4_cr(4) = 0;
    | % -------current vectors completed-------
    | 
    | % create single channel pulsewidth vectors
    | ch1_pw = zeros(1,4)';
    | ch2_pw = zeros(1,4)';
    | ch3_pw = zeros(1,4)';
    | ch4_pw = zeros(1,4)';
    | % assign channel value to first element of each vectors
    | ch1_pw(1) = 1; ch2_pw(1) = 2; ch3_pw(1) = 3; ch4_pw(1) = 4;
    | 
    | % linear map from 0 to max for electrode N
    | slope_north = threshold_max(1)/(integrator_max/2);
    | % linear map from 0 to max for electrode S
    | slope_south = threshold_max(2)/(integrator_max/2);
    | 
    | if (0 <= input_emg)
    |     ch1_pw(2) = abs(slope_north*input_emg);
    |     ch2_pw(2) = 0;
    |     ch3_pw(2) = 0;
    |     ch4_pw(2) = 0;
    | elseif (0 > input_emg)
    |     ch1_pw(2) = 0;
    |     ch2_pw(2) = abs(slope_south*input_emg);
    |     ch3_pw(2) = 0;
    |     ch4_pw(2) = 0;
    | end
    | 
    | % calculate total charge to balance for each channel
    | c2b_ch1 = abs(ch1_pw(2)*stimcr);
    | c2b_ch2 = abs(ch2_pw(2)*stimcr);
    | c2b_ch3 = abs(ch3_pw(2)*stimcr);
    | c2b_ch4 = abs(ch4_pw(2)*stimcr);
    | % calculate and assign balancepw
    | ch1_pw(3) = c2b_ch1/abs(balancecr);
    | ch2_pw(3) = c2b_ch2/abs(balancecr);
    | ch3_pw(3) = c2b_ch3/abs(balancecr);
    | ch4_pw(3) = c2b_ch4/abs(balancecr);
    | % assign pausepw
    | ch1_pw(4) = pausepw; ch2_pw(4) = pausepw; ch3_pw(4) = pausepw; ch4_pw(4) = pausepw;
    | % create null vectors for current and pulsewidth
    | null_ch1 = zeros(1,4)'; null_ch1(1) = 1;
    | null_ch2 = zeros(1,4)'; null_ch2(1) = 2;
    | null_ch3 = zeros(1,4)'; null_ch3(1) = 3;
    | null_ch4 = zeros(1,4)'; null_ch4(1) = 4;
    | 
    | % create output matrices depending on select_channel and select_output
    | if(strcmp('pw',select_output))
    |    output = [ch1_pw, ch2_pw, ch3_pw, ch4_pw];
    | elseif(strcmp('cr',select_output))
    |    output = [ch1_cr, ch2_cr, ch3_cr, ch4_cr];
    | elseif (int8(all(eq(threshold_max,zeros(1,4)))) && strcmp('lg',select_output))
    |    output = 0;
    | elseif (int8(~all(eq(threshold_max,zeros(1,4)))) && strcmp('lg',select_output))
    |    output = 1;
    | else
    |     error('Function paramater error, check parameters for spelling, etc.');    
    | end
    | end
  function output = commonElectrode_4ch_forcefeedback(threshold_max,threshold_min,stimcr,balancecr,pausepw,force_feedback_value,integrator_max,select_output):
    | function output = commonElectrode_4ch_forcefeedback(threshold_max,threshold_min,stimcr,balancecr,pausepw,force_feedback_value,integrator_max,select_output)
    | % create single channel current vectors
    | ch1_cr = zeros(1,4)';
    | ch2_cr = zeros(1,4)';
    | ch3_cr = zeros(1,4)';
    | ch4_cr = zeros(1,4)';
    | % assign channel value to first element of each vector
    | ch1_cr(1) = 1; ch2_cr(1)=2; ch3_cr(1)= 3; ch4_cr(1)=4;
    | % assign stimcr,balancecr and pausecr(=0) to every current vector
    | ch1_cr(2) = stimcr; ch2_cr(2) = stimcr; ch3_cr(2) = stimcr; ch4_cr(2) = stimcr;
    | ch1_cr(3) = balancecr; ch2_cr(3) = balancecr; ch3_cr(3) = balancecr; ch4_cr(3) = balancecr;
    | ch1_cr(4) = 0; ch2_cr(4) = 0; ch3_cr(4) = 0; ch4_cr(4) = 0;
    | % -------current vectors completed-------
    | 
    | % create single channel pulsewidth vectors
    | ch1_pw = zeros(1,4)';
    | ch2_pw = zeros(1,4)';
    | ch3_pw = zeros(1,4)';
    | ch4_pw = zeros(1,4)';
    | % assign channel value to first element of each vectors
    | ch1_pw(1) = 1; ch2_pw(1) = 2; ch3_pw(1) = 3; ch4_pw(1) = 4;
    | 
    | % calculate the slope for 2 segments
    | % from W to N to E
    | slope_W = threshold_max(3)/(integrator_max/2);
    | slope_N = threshold_max(1)/(integrator_max/2);
    | slope_E = threshold_max(4)/(integrator_max/2);
    | 
    | 
    | if (0 <= force_feedback_value) && (force_feedback_value < 6)
    |     ch3_pw(2) = threshold_max(3) - slope_W*force_feedback_value;
    |     ch1_pw(2) = slope_N*force_feedback_value;
    |     ch4_pw(2) = 0;
    |     ch2_pw(2) = 0;
    | elseif (6 <= force_feedback_value) && (force_feedback_value <= 12)
    |     ff_m6 = force_feedback_value - 6;
    |     ch3_pw(2) = 0;
    |     ch1_pw(2) = threshold_max(1) - slope_N*ff_m6;
    |     ch4_pw(2) = slope_E*ff_m6;
    |     ch2_pw(2) = 0;
    | end
    | 
    | % calculate total charge to balance for each channel
    | c2b_ch1 = abs(ch1_pw(2)*stimcr);
    | c2b_ch2 = abs(ch2_pw(2)*stimcr);
    | c2b_ch3 = abs(ch3_pw(2)*stimcr);
    | c2b_ch4 = abs(ch4_pw(2)*stimcr);
    | % calculate and assign balancepw
    | ch1_pw(3) = c2b_ch1/abs(balancecr);
    | ch2_pw(3) = c2b_ch2/abs(balancecr);
    | ch3_pw(3) = c2b_ch3/abs(balancecr);
    | ch4_pw(3) = c2b_ch4/abs(balancecr);
    | % assign pausepw
    | ch1_pw(4) = pausepw; ch2_pw(4) = pausepw; ch3_pw(4) = pausepw; ch4_pw(4) = pausepw;
    | % create null vectors for current and pulsewidth
    | null_ch1 = zeros(1,4)'; null_ch1(1) = 1;
    | null_ch2 = zeros(1,4)'; null_ch2(1) = 2;
    | null_ch3 = zeros(1,4)'; null_ch3(1) = 3;
    | null_ch4 = zeros(1,4)'; null_ch4(1) = 4;
    | 
    | % create output matrices depending on select_channel and select_output
    | if(strcmp('pw',select_output))
    |    output = [ch1_pw, ch2_pw, ch3_pw, ch4_pw];
    | elseif(strcmp('cr',select_output))
    |    output = [ch1_cr, ch2_cr, ch3_cr, ch4_cr];
    | elseif (int8(all(eq(threshold_max,zeros(1,4)))) && strcmp('lg',select_output))
    |    output = 0;
    | elseif (int8(~all(eq(threshold_max,zeros(1,4)))) && strcmp('lg',select_output))
    |    output = 1;
    | else
    |     error('Function paramater error, check parameters for spelling, etc.');    
    | end
    | end
